simulink model "vv_casper"  (R2013b)
settings: Solver=ode45  StartTime=0.0  StopTime=10.0  RelTol=1e-3
undefined symbols (not defined in the file or in its folder): pfb_coeff_gen_calc
undefined symbols (not defined in the file): xlfda_numerator
libraries: xbsIndex_r4 x17488, casper_library_delays x78, casper_library_misc x51, dspsigops x32, xps_library x3, xbsReplacements_r4 x2
(part 7 of 164)

== system vv_casper/dec_fir ==
  sync_in : Inport
  real1 : Inport  Port=2
  imag1 : Inport  Port=3
  real2 : Inport  Port=4
  imag2 : Inport  Port=5
  real3 : Inport  Port=6
  imag3 : Inport  Port=7
  real4 : Inport  Port=8
  imag4 : Inport  Port=9
  real5 : Inport  Port=10
  imag5 : Inport  Port=11
  real6 : Inport  Port=12
  imag6 : Inport  Port=13
  real7 : Inport  Port=14
  imag7 : Inport  Port=15
  real8 : Inport  Port=16
  imag8 : Inport  Port=17
  real9 : Inport  Port=18
  imag9 : Inport  Port=19
  real10 : Inport  Port=20
  imag10 : Inport  Port=21
  real11 : Inport  Port=22
  imag11 : Inport  Port=23
  real12 : Inport  Port=24
  imag12 : Inport  Port=25
  real13 : Inport  Port=26
  imag13 : Inport  Port=27
  real14 : Inport  Port=28
  imag14 : Inport  Port=29
  real15 : Inport  Port=30
  imag15 : Inport  Port=31
  real16 : Inport  Port=32
  imag16 : Inport  Port=33
  convert1 : xbsIndex_r4/Convert  gui_display_data_type=Fixed-point  arith_type="Signed  (2's comp)"  n_bits=35  bin_pt=34  float_type=Single  exp_bits=8  fraction_bits=24  quantization="Round  (unbiased: +/- Inf)"  overflow=Wrap  en=off  latency=2  dbl_ovrd=off  pipeline=off  block_type=convert
  convert2 : xbsIndex_r4/Convert  gui_display_data_type=Fixed-point  arith_type="Signed  (2's comp)"  n_bits=35  bin_pt=34  float_type=Single  exp_bits=8  fraction_bits=24  quantization="Round  (unbiased: +/- Inf)"  overflow=Wrap  en=off  latency=2  dbl_ovrd=off  pipeline=off  block_type=convert
  delay : xbsIndex_r4/Delay  rst=off  infoeditControl=Selection of Reset will increase slice count due to use of real FFs and instead of SRLs  en=off  latency=9  dbl_ovrd=off  reg_retiming=off  block_type=delay
  fir_dbl_col1 : Subsystem  AncestorBlock=casper_library_downconverter/fir_dbl_col  mask(fir_dbl_col){n_inputs=16, coeff=[-0.00011716 -9.1991e-05 -6.4266e-05  -3.536e-05 -6.6251e-06  2.0662e-05  4.5356e-05  6.6484e-05  8.3286e-05  9.5227e-05  0.00010202  0.00010362   0.0001002   9.217e-05  8.0098e-05  6.4705e-05], add_latency=1, mult_latency=2, coeff_bit_width=25, coeff_bin_pt=24, first_stage_hdl=on, adder_imp=DSP48}
      mask prompts: n_inputs "Inputs"; coeff "Coefficients"; add_latency "Add latency"; mult_latency "Mult Latency"; coeff_bit_width "Coefficient bit width"; coeff_bin_pt "Coefficient binary point"; first_stage_hdl "Implement first stage of adder trees on output as behavioural HDL"; adder_imp "Adder implementation"
      mask init:
      | fir_dbl_col_init(gcb, ...
      |     'n_inputs', n_inputs, ...
      |     'coeff', coeff, ...
      |     'mult_latency', mult_latency, ...
      |     'add_latency', add_latency, ...
      |     'coeff_bit_width', coeff_bit_width, ...
      |     'coeff_bin_pt', coeff_bin_pt,  ...
      |     'first_stage_hdl', first_stage_hdl, ...
      |     'adder_imp', adder_imp);
      mask Help: eval('xlWeb(''http://casper.berkeley.edu/wiki/Fir_dbl_col'')')
      mask TypeOptions adder_imp: Behavioral | Fabric | DSP48
  fir_dbl_col10 : Subsystem  AncestorBlock=casper_library_downconverter/fir_dbl_col  mask(fir_dbl_col){n_inputs=16, coeff=[0.0019945   0.0022285   0.0023628   0.0023951   0.0023272   0.0021652   0.0019186   0.0016003   0.0012258  0.00081224    0.000378 -5.8305e-05 -0.00047857 -0.00086589  -0.0012053  -0.0014841], add_latency=1, mult_latency=2, coeff_bit_width=25, coeff_bin_pt=24, first_stage_hdl=on, adder_imp=DSP48}
      mask prompts: n_inputs "Inputs"; coeff "Coefficients"; add_latency "Add latency"; mult_latency "Mult Latency"; coeff_bit_width "Coefficient bit width"; coeff_bin_pt "Coefficient binary point"; first_stage_hdl "Implement first stage of adder trees on output as behavioural HDL"; adder_imp "Adder implementation"
      mask init: same as vv_casper/dec_fir/fir_dbl_col1
      mask Help: eval('xlWeb(''http://casper.berkeley.edu/wiki/Fir_dbl_col'')')
      mask TypeOptions adder_imp: Behavioral | Fabric | DSP48
  fir_dbl_col11 : Subsystem  AncestorBlock=casper_library_downconverter/fir_dbl_col  mask(fir_dbl_col){n_inputs=16, coeff=[-0.0023054  -0.0026857  -0.0029423  -0.0030687  -0.0030641  -0.0029331  -0.0026851  -0.0023343  -0.0018984  -0.0013982 -0.00085648 -0.00029684  0.00025703  0.00078246   0.0012587   0.0016676], add_latency=1, mult_latency=2, coeff_bit_width=25, coeff_bin_pt=24, first_stage_hdl=on, adder_imp=DSP48}
      mask prompts: n_inputs "Inputs"; coeff "Coefficients"; add_latency "Add latency"; mult_latency "Mult Latency"; coeff_bit_width "Coefficient bit width"; coeff_bin_pt "Coefficient binary point"; first_stage_hdl "Implement first stage of adder trees on output as behavioural HDL"; adder_imp "Adder implementation"
      mask init: same as vv_casper/dec_fir/fir_dbl_col1
      mask Help: eval('xlWeb(''http://casper.berkeley.edu/wiki/Fir_dbl_col'')')
      mask TypeOptions adder_imp: Behavioral | Fabric | DSP48
  fir_dbl_col12 : Subsystem  AncestorBlock=casper_library_downconverter/fir_dbl_col  mask(fir_dbl_col){n_inputs=16, coeff=[0.0026286   0.0032244    0.003665   0.0039383   0.0040391   0.0039697   0.0037391   0.0033626   0.0028607   0.0022586   0.0015845  0.00086849   0.0001415 -0.00056625  -0.0012263  -0.0018133], add_latency=1, mult_latency=2, coeff_bit_width=25, coeff_bin_pt=24, first_stage_hdl=on, adder_imp=DSP48}
      mask prompts: n_inputs "Inputs"; coeff "Coefficients"; add_latency "Add latency"; mult_latency "Mult Latency"; coeff_bit_width "Coefficient bit width"; coeff_bin_pt "Coefficient binary point"; first_stage_hdl "Implement first stage of adder trees on output as behavioural HDL"; adder_imp "Adder implementation"
      mask init: same as vv_casper/dec_fir/fir_dbl_col1
      mask Help: eval('xlWeb(''http://casper.berkeley.edu/wiki/Fir_dbl_col'')')
      mask TypeOptions adder_imp: Behavioral | Fabric | DSP48
  fir_dbl_col13 : Subsystem  AncestorBlock=casper_library_downconverter/fir_dbl_col  mask(fir_dbl_col){n_inputs=16, coeff=[-0.0029853  -0.0039218  -0.0046552  -0.0051649  -0.0054403  -0.0054803  -0.0052935  -0.0048969  -0.0043155  -0.0035804  -0.0027279  -0.0017974 -0.00082976  0.00013403   0.0010549   0.0018968], add_latency=1, mult_latency=2, coeff_bit_width=25, coeff_bin_pt=24, first_stage_hdl=on, adder_imp=DSP48}
      mask prompts: n_inputs "Inputs"; coeff "Coefficients"; add_latency "Add latency"; mult_latency "Mult Latency"; coeff_bit_width "Coefficient bit width"; coeff_bin_pt "Coefficient binary point"; first_stage_hdl "Implement first stage of adder trees on output as behavioural HDL"; adder_imp "Adder implementation"
      mask init: same as vv_casper/dec_fir/fir_dbl_col1
      mask Help: eval('xlWeb(''http://casper.berkeley.edu/wiki/Fir_dbl_col'')')
      mask TypeOptions adder_imp: Behavioral | Fabric | DSP48
  fir_dbl_col14 : Subsystem  AncestorBlock=casper_library_downconverter/fir_dbl_col  mask(fir_dbl_col){n_inputs=16, coeff=[0.0034602   0.0050242   0.0062876   0.0072191    0.007802   0.0080335   0.0079243   0.0074975   0.0067875   0.0058373   0.0046975   0.0034231   0.0020719  0.00070185 -0.00063127  -0.0018756], add_latency=1, mult_latency=2, coeff_bit_width=25, coeff_bin_pt=24, first_stage_hdl=on, adder_imp=DSP48}
      mask prompts: n_inputs "Inputs"; coeff "Coefficients"; add_latency "Add latency"; mult_latency "Mult Latency"; coeff_bit_width "Coefficient bit width"; coeff_bin_pt "Coefficient binary point"; first_stage_hdl "Implement first stage of adder trees on output as behavioural HDL"; adder_imp "Adder implementation"
      mask init: same as vv_casper/dec_fir/fir_dbl_col1
      mask Help: eval('xlWeb(''http://casper.berkeley.edu/wiki/Fir_dbl_col'')')
      mask TypeOptions adder_imp: Behavioral | Fabric | DSP48
  fir_dbl_col15 : Subsystem  AncestorBlock=casper_library_downconverter/fir_dbl_col  mask(fir_dbl_col){n_inputs=16, coeff=[-0.004503  -0.0077173   -0.010272   -0.012152    -0.01336   -0.013919    -0.01387   -0.013269   -0.012184   -0.010697  -0.0088951  -0.0068697  -0.0047146  -0.0025212 -0.00037637   0.0016407], add_latency=1, mult_latency=2, coeff_bit_width=25, coeff_bin_pt=24, first_stage_hdl=on, adder_imp=DSP48}
      mask prompts: n_inputs "Inputs"; coeff "Coefficients"; add_latency "Add latency"; mult_latency "Mult Latency"; coeff_bit_width "Coefficient bit width"; coeff_bin_pt "Coefficient binary point"; first_stage_hdl "Implement first stage of adder trees on output as behavioural HDL"; adder_imp "Adder implementation"
      mask init: same as vv_casper/dec_fir/fir_dbl_col1
      mask Help: eval('xlWeb(''http://casper.berkeley.edu/wiki/Fir_dbl_col'')')
      mask TypeOptions adder_imp: Behavioral | Fabric | DSP48
  fir_dbl_col16 : Subsystem  AncestorBlock=casper_library_downconverter/fir_dbl_col  mask(fir_dbl_col){n_inputs=16, coeff=[0.065072    0.064162    0.062365    0.059726    0.056312    0.052207    0.047514    0.042348    0.036834    0.031102    0.025287    0.019521     0.01393    0.008634    0.003738 -0.00066588], add_latency=1, mult_latency=2, coeff_bit_width=25, coeff_bin_pt=24, first_stage_hdl=on, adder_imp=DSP48}
      mask prompts: n_inputs "Inputs"; coeff "Coefficients"; add_latency "Add latency"; mult_latency "Mult Latency"; coeff_bit_width "Coefficient bit width"; coeff_bin_pt "Coefficient binary point"; first_stage_hdl "Implement first stage of adder trees on output as behavioural HDL"; adder_imp "Adder implementation"
      mask init: same as vv_casper/dec_fir/fir_dbl_col1
      mask Help: eval('xlWeb(''http://casper.berkeley.edu/wiki/Fir_dbl_col'')')
      mask TypeOptions adder_imp: Behavioral | Fabric | DSP48
  fir_dbl_col2 : Subsystem  AncestorBlock=casper_library_downconverter/fir_dbl_col  mask(fir_dbl_col){n_inputs=16, coeff=[0.00020848  0.00017636  0.00013837  9.6442e-05  5.2572e-05  8.7473e-06 -3.3147e-05   -7.14e-05 -0.00010455 -0.00013141 -0.00015117 -0.00016332 -0.00016775 -0.00016468 -0.00015464 -0.00013845], add_latency=1, mult_latency=2, coeff_bit_width=25, coeff_bin_pt=24, first_stage_hdl=on, adder_imp=DSP48}
      mask prompts: n_inputs "Inputs"; coeff "Coefficients"; add_latency "Add latency"; mult_latency "Mult Latency"; coeff_bit_width "Coefficient bit width"; coeff_bin_pt "Coefficient binary point"; first_stage_hdl "Implement first stage of adder trees on output as behavioural HDL"; adder_imp "Adder implementation"
      mask init: same as vv_casper/dec_fir/fir_dbl_col1
      mask Help: eval('xlWeb(''http://casper.berkeley.edu/wiki/Fir_dbl_col'')')
      mask TypeOptions adder_imp: Behavioral | Fabric | DSP48
  fir_dbl_col3 : Subsystem  AncestorBlock=casper_library_downconverter/fir_dbl_col  mask(fir_dbl_col){n_inputs=16, coeff=[-0.00032924 -0.00029221 -0.00024455 -0.00018874 -0.00012752 -6.3715e-05  -1.479e-07  6.0493e-05  0.00011577  0.00016357  0.00020222  0.00023048  0.00024766  0.00025353   0.0002484  0.00023299], add_latency=1, mult_latency=2, coeff_bit_width=25, coeff_bin_pt=24, first_stage_hdl=on, adder_imp=DSP48}
      mask prompts: n_inputs "Inputs"; coeff "Coefficients"; add_latency "Add latency"; mult_latency "Mult Latency"; coeff_bit_width "Coefficient bit width"; coeff_bin_pt "Coefficient binary point"; first_stage_hdl "Implement first stage of adder trees on output as behavioural HDL"; adder_imp "Adder implementation"
      mask init: same as vv_casper/dec_fir/fir_dbl_col1
      mask Help: eval('xlWeb(''http://casper.berkeley.edu/wiki/Fir_dbl_col'')')
      mask TypeOptions adder_imp: Behavioral | Fabric | DSP48
  fir_dbl_col4 : Subsystem  AncestorBlock=casper_library_downconverter/fir_dbl_col  mask(fir_dbl_col){n_inputs=16, coeff=[0.00048235  0.00044471  0.00038999  0.00032117   0.0002417  0.00015536  6.6049e-05 -2.2349e-05 -0.00010615 -0.00018201 -0.00024707 -0.00029904 -0.00033626 -0.00035779  -0.0003634 -0.00035352], add_latency=1, mult_latency=2, coeff_bit_width=25, coeff_bin_pt=24, first_stage_hdl=on, adder_imp=DSP48}
      mask prompts: n_inputs "Inputs"; coeff "Coefficients"; add_latency "Add latency"; mult_latency "Mult Latency"; coeff_bit_width "Coefficient bit width"; coeff_bin_pt "Coefficient binary point"; first_stage_hdl "Implement first stage of adder trees on output as behavioural HDL"; adder_imp "Adder implementation"
      mask init: same as vv_casper/dec_fir/fir_dbl_col1
      mask Help: eval('xlWeb(''http://casper.berkeley.edu/wiki/Fir_dbl_col'')')
      mask TypeOptions adder_imp: Behavioral | Fabric | DSP48
  fir_dbl_col5 : Subsystem  AncestorBlock=casper_library_downconverter/fir_dbl_col  mask(fir_dbl_col){n_inputs=16, coeff=[-0.00066852 -0.00063712 -0.00058034 -0.00050146  -0.0004046 -0.00029448 -0.00017619 -5.4992e-05  6.3927e-05  0.00017567  0.00027583  0.00036064  0.00042714  0.00047323  0.00049777  0.00050057], add_latency=1, mult_latency=2, coeff_bit_width=25, coeff_bin_pt=24, first_stage_hdl=on, adder_imp=DSP48}
      mask prompts: n_inputs "Inputs"; coeff "Coefficients"; add_latency "Add latency"; mult_latency "Mult Latency"; coeff_bit_width "Coefficient bit width"; coeff_bin_pt "Coefficient binary point"; first_stage_hdl "Implement first stage of adder trees on output as behavioural HDL"; adder_imp "Adder implementation"
      mask init: same as vv_casper/dec_fir/fir_dbl_col1
      mask Help: eval('xlWeb(''http://casper.berkeley.edu/wiki/Fir_dbl_col'')')
      mask TypeOptions adder_imp: Behavioral | Fabric | DSP48
  fir_dbl_col6 : Subsystem  AncestorBlock=casper_library_downconverter/fir_dbl_col  mask(fir_dbl_col){n_inputs=16, coeff=[0.00088649   0.0008712  0.00082022  0.00073687  0.00062575  0.00049244  0.00034327  0.00018502  2.4603e-05  -0.0001312 -0.00027605 -0.00040428 -0.00051111 -0.00059285 -0.00064697  -0.0006722], add_latency=1, mult_latency=2, coeff_bit_width=25, coeff_bin_pt=24, first_stage_hdl=on, adder_imp=DSP48}
      mask prompts: n_inputs "Inputs"; coeff "Coefficients"; add_latency "Add latency"; mult_latency "Mult Latency"; coeff_bit_width "Coefficient bit width"; coeff_bin_pt "Coefficient binary point"; first_stage_hdl "Implement first stage of adder trees on output as behavioural HDL"; adder_imp "Adder implementation"
      mask init: same as vv_casper/dec_fir/fir_dbl_col1
      mask Help: eval('xlWeb(''http://casper.berkeley.edu/wiki/Fir_dbl_col'')')
      mask TypeOptions adder_imp: Behavioral | Fabric | DSP48
  fir_dbl_col7 : Subsystem  AncestorBlock=casper_library_downconverter/fir_dbl_col  mask(fir_dbl_col){n_inputs=16, coeff=[-0.0011332  -0.0011474  -0.0011135  -0.0010345 -0.00091512 -0.00076162 -0.00058152  -0.0003832  -0.0001755  3.2606e-05  0.00023245  0.00041597  0.00057606  0.00070685  0.00080384  0.00086415], add_latency=1, mult_latency=2, coeff_bit_width=25, coeff_bin_pt=24, first_stage_hdl=on, adder_imp=DSP48}
      mask prompts: n_inputs "Inputs"; coeff "Coefficients"; add_latency "Add latency"; mult_latency "Mult Latency"; coeff_bit_width "Coefficient bit width"; coeff_bin_pt "Coefficient binary point"; first_stage_hdl "Implement first stage of adder trees on output as behavioural HDL"; adder_imp "Adder implementation"
      mask init: same as vv_casper/dec_fir/fir_dbl_col1
      mask Help: eval('xlWeb(''http://casper.berkeley.edu/wiki/Fir_dbl_col'')')
      mask TypeOptions adder_imp: Behavioral | Fabric | DSP48
  fir_dbl_col8 : Subsystem  AncestorBlock=casper_library_downconverter/fir_dbl_col  mask(fir_dbl_col){n_inputs=16, coeff=[0.0014038   0.0014653   0.0014641   0.0014022    0.001284   0.0011164  0.00090766  0.00066792  0.00040807  0.00013955 -0.00012621 -0.00037824 -0.00060651 -0.00080228 -0.00095846  -0.0010698], add_latency=1, mult_latency=2, coeff_bit_width=25, coeff_bin_pt=24, first_stage_hdl=on, adder_imp=DSP48}
      mask prompts: n_inputs "Inputs"; coeff "Coefficients"; add_latency "Add latency"; mult_latency "Mult Latency"; coeff_bit_width "Coefficient bit width"; coeff_bin_pt "Coefficient binary point"; first_stage_hdl "Implement first stage of adder trees on output as behavioural HDL"; adder_imp "Adder implementation"
      mask init: same as vv_casper/dec_fir/fir_dbl_col1
      mask Help: eval('xlWeb(''http://casper.berkeley.edu/wiki/Fir_dbl_col'')')
      mask TypeOptions adder_imp: Behavioral | Fabric | DSP48
  fir_dbl_col9 : Subsystem  AncestorBlock=casper_library_downconverter/fir_dbl_col  mask(fir_dbl_col){n_inputs=16, coeff=[-0.0016928  -0.0018249  -0.0018772  -0.0018501  -0.0017472  -0.0015751  -0.0013431  -0.0010626 -0.00074681 -0.00040991 -6.6527e-05   0.0002689   0.0005827  0.00086252   0.0010978   0.0012802], add_latency=1, mult_latency=2, coeff_bit_width=25, coeff_bin_pt=24, first_stage_hdl=on, adder_imp=DSP48}
      mask prompts: n_inputs "Inputs"; coeff "Coefficients"; add_latency "Add latency"; mult_latency "Mult Latency"; coeff_bit_width "Coefficient bit width"; coeff_bin_pt "Coefficient binary point"; first_stage_hdl "Implement first stage of adder trees on output as behavioural HDL"; adder_imp "Adder implementation"
      mask init: same as vv_casper/dec_fir/fir_dbl_col1
      mask Help: eval('xlWeb(''http://casper.berkeley.edu/wiki/Fir_dbl_col'')')
      mask TypeOptions adder_imp: Behavioral | Fabric | DSP48
  imag_sum : Subsystem  AncestorBlock=casper_library_misc/adder_tree  mask(adder_tree){n_inputs=16, latency=1, adder_imp=DSP48, first_stage_hdl=off}
      mask prompts: n_inputs "Number of Inputs"; latency "Add Latency"; adder_imp "Adder implementation"; first_stage_hdl "Use behavioural HDL for first stage of adders"
      mask help:
      | Sums all inputs using a tree of adds and delays.
      |
      | Number of inputs: The number of inputs to the block to be summed
      | Add latency: The number of clock cycles to perform one addition (affects timing)..
      | Adder implementation: choice of fabric or DSP48E core, or behavioral HDL
      | Use behavioural HDL for first stage of adders: Causes the first stage of adders to be absorbed into DSP blocks if multipliers precede them (Virtex 5). Overrides Adder implementation
      mask init:
      | adder_tree_init(gcb, ...
      |     'n_inputs', n_inputs, ...
      |     'latency', latency, ...
      |     'adder_imp', adder_imp, ...
      |     'first_stage_hdl', first_stage_hdl);
      settings: AttributesFormatString=latency 4
      mask Help: eval('xlWeb(''http://casper.berkeley.edu/wiki/Adder_tree'')')
      mask TypeOptions adder_imp: Behavioral | Fabric | DSP48
  real_sum : Subsystem  AncestorBlock=casper_library_misc/adder_tree  mask(adder_tree){n_inputs=16, latency=1, adder_imp=DSP48, first_stage_hdl=off}
      mask prompts: n_inputs "Number of Inputs"; latency "Add Latency"; adder_imp "Adder implementation"; first_stage_hdl "Use behavioural HDL for first stage of adders"
      mask help:
      | Sums all inputs using a tree of adds and delays.
      |
      | Number of inputs: The number of inputs to the block to be summed
      | Add latency: The number of clock cycles to perform one addition (affects timing)..
      | Adder implementation: choice of fabric or DSP48E core, or behavioral HDL
      | Use behavioural HDL for first stage of adders: Causes the first stage of adders to be absorbed into DSP blocks if multipliers precede them (Virtex 5). Overrides Adder implementation
      mask init:
      | adder_tree_init(gcb, ...
      |     'n_inputs', n_inputs, ...
      |     'latency', latency, ...
      |     'adder_imp', adder_imp, ...
      |     'first_stage_hdl', first_stage_hdl);
      settings: AttributesFormatString=latency 4
      mask Help: eval('xlWeb(''http://casper.berkeley.edu/wiki/Adder_tree'')')
      mask TypeOptions adder_imp: Behavioral | Fabric | DSP48
  ri_to_c : casper_library_misc/ri_to_c
  shift1 : xbsIndex_r4/Shift  shift_dir=Left  shift_bits=0  en=off  latency=0  precision=Full  arith_type="Signed  (2's comp)"  n_bits=16  bin_pt=14  quantization=Truncate  overflow=Wrap  dbl_ovrd=off  block_type=shift
  shift2 : xbsIndex_r4/Shift  shift_dir=Left  shift_bits=0  en=off  latency=0  precision=Full  arith_type="Signed  (2's comp)"  n_bits=16  bin_pt=14  quantization=Truncate  overflow=Wrap  dbl_ovrd=off  block_type=shift
  sync_out : Outport
  dout : Outport  Port=2
  wires:
  real1/1 -> fir_dbl_col1/1(real1)
  imag1/1 -> fir_dbl_col1/2(imag1)
  real2/1 -> fir_dbl_col1/3(real2)
  imag2/1 -> fir_dbl_col1/4(imag2)
  real3/1 -> fir_dbl_col1/5(real3)
  imag3/1 -> fir_dbl_col1/6(imag3)
  real4/1 -> fir_dbl_col1/7(real4)
  imag4/1 -> fir_dbl_col1/8(imag4)
  real5/1 -> fir_dbl_col1/9(real5)
  imag5/1 -> fir_dbl_col1/10(imag5)
  real6/1 -> fir_dbl_col1/11(real6)
  imag6/1 -> fir_dbl_col1/12(imag6)
  real7/1 -> fir_dbl_col1/13(real7)
  imag7/1 -> fir_dbl_col1/14(imag7)
  real8/1 -> fir_dbl_col1/15(real8)
  imag8/1 -> fir_dbl_col1/16(imag8)
  real9/1 -> fir_dbl_col1/17(real9)
  imag9/1 -> fir_dbl_col1/18(imag9)
  real10/1 -> fir_dbl_col1/19(real10)
  imag10/1 -> fir_dbl_col1/20(imag10)
  real11/1 -> fir_dbl_col1/21(real11)
  imag11/1 -> fir_dbl_col1/22(imag11)
  real12/1 -> fir_dbl_col1/23(real12)
  imag12/1 -> fir_dbl_col1/24(imag12)
  real13/1 -> fir_dbl_col1/25(real13)
  imag13/1 -> fir_dbl_col1/26(imag13)
  real14/1 -> fir_dbl_col1/27(real14)
  imag14/1 -> fir_dbl_col1/28(imag14)
  real15/1 -> fir_dbl_col1/29(real15)
  imag15/1 -> fir_dbl_col1/30(imag15)
  real16/1 -> fir_dbl_col1/31(real16)
  imag16/1 -> fir_dbl_col1/32(imag16)
  fir_dbl_col1/65(real_sum) -> real_sum/2(din1)
  fir_dbl_col1/66(imag_sum) -> imag_sum/2(din1)
  fir_dbl_col1/1(real_out1) -> fir_dbl_col2/1(real1)
  fir_dbl_col1/2(imag_out1) -> fir_dbl_col2/2(imag1)
  fir_dbl_col1/3(real_out2) -> fir_dbl_col2/3(real2)
  fir_dbl_col1/4(imag_out2) -> fir_dbl_col2/4(imag2)
  fir_dbl_col1/5(real_out3) -> fir_dbl_col2/5(real3)
  fir_dbl_col1/6(imag_out3) -> fir_dbl_col2/6(imag3)
  fir_dbl_col1/7(real_out4) -> fir_dbl_col2/7(real4)
  fir_dbl_col1/8(imag_out4) -> fir_dbl_col2/8(imag4)
  fir_dbl_col1/9(real_out5) -> fir_dbl_col2/9(real5)
  fir_dbl_col1/10(imag_out5) -> fir_dbl_col2/10(imag5)
  fir_dbl_col1/11(real_out6) -> fir_dbl_col2/11(real6)
  fir_dbl_col1/12(imag_out6) -> fir_dbl_col2/12(imag6)
  fir_dbl_col1/13(real_out7) -> fir_dbl_col2/13(real7)
  fir_dbl_col1/14(imag_out7) -> fir_dbl_col2/14(imag7)
  fir_dbl_col1/15(real_out8) -> fir_dbl_col2/15(real8)
  fir_dbl_col1/16(imag_out8) -> fir_dbl_col2/16(imag8)
  fir_dbl_col1/17(real_out9) -> fir_dbl_col2/17(real9)
  fir_dbl_col1/18(imag_out9) -> fir_dbl_col2/18(imag9)
  fir_dbl_col1/19(real_out10) -> fir_dbl_col2/19(real10)
  fir_dbl_col1/20(imag_out10) -> fir_dbl_col2/20(imag10)
  fir_dbl_col1/21(real_out11) -> fir_dbl_col2/21(real11)
  fir_dbl_col1/22(imag_out11) -> fir_dbl_col2/22(imag11)
  fir_dbl_col1/23(real_out12) -> fir_dbl_col2/23(real12)
  fir_dbl_col1/24(imag_out12) -> fir_dbl_col2/24(imag12)
  fir_dbl_col1/25(real_out13) -> fir_dbl_col2/25(real13)
  fir_dbl_col1/26(imag_out13) -> fir_dbl_col2/26(imag13)
  fir_dbl_col1/27(real_out14) -> fir_dbl_col2/27(real14)
  fir_dbl_col1/28(imag_out14) -> fir_dbl_col2/28(imag14)
  fir_dbl_col1/29(real_out15) -> fir_dbl_col2/29(real15)
  fir_dbl_col1/30(imag_out15) -> fir_dbl_col2/30(imag15)
  fir_dbl_col1/31(real_out16) -> fir_dbl_col2/31(real16)
  fir_dbl_col1/32(imag_out16) -> fir_dbl_col2/32(imag16)
  fir_dbl_col2/65(real_sum) -> real_sum/3(din2)
  fir_dbl_col2/66(imag_sum) -> imag_sum/3(din2)
  fir_dbl_col2/1(real_out1) -> fir_dbl_col3/1(real1)
  fir_dbl_col2/2(imag_out1) -> fir_dbl_col3/2(imag1)
  fir_dbl_col2/3(real_out2) -> fir_dbl_col3/3(real2)
  fir_dbl_col2/4(imag_out2) -> fir_dbl_col3/4(imag2)
  fir_dbl_col2/5(real_out3) -> fir_dbl_col3/5(real3)
  fir_dbl_col2/6(imag_out3) -> fir_dbl_col3/6(imag3)
  fir_dbl_col2/7(real_out4) -> fir_dbl_col3/7(real4)
  fir_dbl_col2/8(imag_out4) -> fir_dbl_col3/8(imag4)
  fir_dbl_col2/9(real_out5) -> fir_dbl_col3/9(real5)
  fir_dbl_col2/10(imag_out5) -> fir_dbl_col3/10(imag5)
  fir_dbl_col2/11(real_out6) -> fir_dbl_col3/11(real6)
  fir_dbl_col2/12(imag_out6) -> fir_dbl_col3/12(imag6)
  fir_dbl_col2/13(real_out7) -> fir_dbl_col3/13(real7)
  fir_dbl_col2/14(imag_out7) -> fir_dbl_col3/14(imag7)
  fir_dbl_col2/15(real_out8) -> fir_dbl_col3/15(real8)
  fir_dbl_col2/16(imag_out8) -> fir_dbl_col3/16(imag8)
  fir_dbl_col2/17(real_out9) -> fir_dbl_col3/17(real9)
  fir_dbl_col2/18(imag_out9) -> fir_dbl_col3/18(imag9)
  fir_dbl_col2/19(real_out10) -> fir_dbl_col3/19(real10)
  fir_dbl_col2/20(imag_out10) -> fir_dbl_col3/20(imag10)
  fir_dbl_col2/21(real_out11) -> fir_dbl_col3/21(real11)
  fir_dbl_col2/22(imag_out11) -> fir_dbl_col3/22(imag11)
  fir_dbl_col2/23(real_out12) -> fir_dbl_col3/23(real12)
  fir_dbl_col2/24(imag_out12) -> fir_dbl_col3/24(imag12)
  fir_dbl_col2/25(real_out13) -> fir_dbl_col3/25(real13)
  fir_dbl_col2/26(imag_out13) -> fir_dbl_col3/26(imag13)
  fir_dbl_col2/27(real_out14) -> fir_dbl_col3/27(real14)
  fir_dbl_col2/28(imag_out14) -> fir_dbl_col3/28(imag14)
  fir_dbl_col2/29(real_out15) -> fir_dbl_col3/29(real15)
  fir_dbl_col2/30(imag_out15) -> fir_dbl_col3/30(imag15)
  fir_dbl_col2/31(real_out16) -> fir_dbl_col3/31(real16)
  fir_dbl_col2/32(imag_out16) -> fir_dbl_col3/32(imag16)
  fir_dbl_col3/65(real_sum) -> real_sum/4(din3)
  fir_dbl_col3/66(imag_sum) -> imag_sum/4(din3)
  fir_dbl_col3/1(real_out1) -> fir_dbl_col4/1(real1)
  fir_dbl_col3/2(imag_out1) -> fir_dbl_col4/2(imag1)
  fir_dbl_col3/3(real_out2) -> fir_dbl_col4/3(real2)
  fir_dbl_col3/4(imag_out2) -> fir_dbl_col4/4(imag2)
  fir_dbl_col3/5(real_out3) -> fir_dbl_col4/5(real3)
  fir_dbl_col3/6(imag_out3) -> fir_dbl_col4/6(imag3)
  fir_dbl_col3/7(real_out4) -> fir_dbl_col4/7(real4)
  fir_dbl_col3/8(imag_out4) -> fir_dbl_col4/8(imag4)
  fir_dbl_col3/9(real_out5) -> fir_dbl_col4/9(real5)
  fir_dbl_col3/10(imag_out5) -> fir_dbl_col4/10(imag5)
  fir_dbl_col3/11(real_out6) -> fir_dbl_col4/11(real6)
  fir_dbl_col3/12(imag_out6) -> fir_dbl_col4/12(imag6)
  fir_dbl_col3/13(real_out7) -> fir_dbl_col4/13(real7)
  fir_dbl_col3/14(imag_out7) -> fir_dbl_col4/14(imag7)
  fir_dbl_col3/15(real_out8) -> fir_dbl_col4/15(real8)
  fir_dbl_col3/16(imag_out8) -> fir_dbl_col4/16(imag8)
  fir_dbl_col3/17(real_out9) -> fir_dbl_col4/17(real9)
  fir_dbl_col3/18(imag_out9) -> fir_dbl_col4/18(imag9)
  fir_dbl_col3/19(real_out10) -> fir_dbl_col4/19(real10)
  fir_dbl_col3/20(imag_out10) -> fir_dbl_col4/20(imag10)
  fir_dbl_col3/21(real_out11) -> fir_dbl_col4/21(real11)
  fir_dbl_col3/22(imag_out11) -> fir_dbl_col4/22(imag11)
  fir_dbl_col3/23(real_out12) -> fir_dbl_col4/23(real12)
  fir_dbl_col3/24(imag_out12) -> fir_dbl_col4/24(imag12)
  fir_dbl_col3/25(real_out13) -> fir_dbl_col4/25(real13)
  fir_dbl_col3/26(imag_out13) -> fir_dbl_col4/26(imag13)
  fir_dbl_col3/27(real_out14) -> fir_dbl_col4/27(real14)
  fir_dbl_col3/28(imag_out14) -> fir_dbl_col4/28(imag14)
  fir_dbl_col3/29(real_out15) -> fir_dbl_col4/29(real15)
  fir_dbl_col3/30(imag_out15) -> fir_dbl_col4/30(imag15)
  fir_dbl_col3/31(real_out16) -> fir_dbl_col4/31(real16)
  fir_dbl_col3/32(imag_out16) -> fir_dbl_col4/32(imag16)
  fir_dbl_col4/65(real_sum) -> real_sum/5(din4)
  fir_dbl_col4/66(imag_sum) -> imag_sum/5(din4)
  fir_dbl_col4/1(real_out1) -> fir_dbl_col5/1(real1)
  fir_dbl_col4/2(imag_out1) -> fir_dbl_col5/2(imag1)
  fir_dbl_col4/3(real_out2) -> fir_dbl_col5/3(real2)
  fir_dbl_col4/4(imag_out2) -> fir_dbl_col5/4(imag2)
  fir_dbl_col4/5(real_out3) -> fir_dbl_col5/5(real3)
  fir_dbl_col4/6(imag_out3) -> fir_dbl_col5/6(imag3)
  fir_dbl_col4/7(real_out4) -> fir_dbl_col5/7(real4)
  fir_dbl_col4/8(imag_out4) -> fir_dbl_col5/8(imag4)
  fir_dbl_col4/9(real_out5) -> fir_dbl_col5/9(real5)
  fir_dbl_col4/10(imag_out5) -> fir_dbl_col5/10(imag5)
  fir_dbl_col4/11(real_out6) -> fir_dbl_col5/11(real6)
  fir_dbl_col4/12(imag_out6) -> fir_dbl_col5/12(imag6)
  fir_dbl_col4/13(real_out7) -> fir_dbl_col5/13(real7)
  fir_dbl_col4/14(imag_out7) -> fir_dbl_col5/14(imag7)
  fir_dbl_col4/15(real_out8) -> fir_dbl_col5/15(real8)
  fir_dbl_col4/16(imag_out8) -> fir_dbl_col5/16(imag8)
  fir_dbl_col4/17(real_out9) -> fir_dbl_col5/17(real9)
  fir_dbl_col4/18(imag_out9) -> fir_dbl_col5/18(imag9)
  fir_dbl_col4/19(real_out10) -> fir_dbl_col5/19(real10)
  fir_dbl_col4/20(imag_out10) -> fir_dbl_col5/20(imag10)
  fir_dbl_col4/21(real_out11) -> fir_dbl_col5/21(real11)
  fir_dbl_col4/22(imag_out11) -> fir_dbl_col5/22(imag11)
  fir_dbl_col4/23(real_out12) -> fir_dbl_col5/23(real12)
  fir_dbl_col4/24(imag_out12) -> fir_dbl_col5/24(imag12)
  fir_dbl_col4/25(real_out13) -> fir_dbl_col5/25(real13)
  fir_dbl_col4/26(imag_out13) -> fir_dbl_col5/26(imag13)
  fir_dbl_col4/27(real_out14) -> fir_dbl_col5/27(real14)
  fir_dbl_col4/28(imag_out14) -> fir_dbl_col5/28(imag14)
  fir_dbl_col4/29(real_out15) -> fir_dbl_col5/29(real15)
  fir_dbl_col4/30(imag_out15) -> fir_dbl_col5/30(imag15)
  fir_dbl_col4/31(real_out16) -> fir_dbl_col5/31(real16)
  fir_dbl_col4/32(imag_out16) -> fir_dbl_col5/32(imag16)
  fir_dbl_col5/65(real_sum) -> real_sum/6(din5)
  fir_dbl_col5/66(imag_sum) -> imag_sum/6(din5)
  fir_dbl_col5/1(real_out1) -> fir_dbl_col6/1(real1)
  fir_dbl_col5/2(imag_out1) -> fir_dbl_col6/2(imag1)
  fir_dbl_col5/3(real_out2) -> fir_dbl_col6/3(real2)
  fir_dbl_col5/4(imag_out2) -> fir_dbl_col6/4(imag2)
  fir_dbl_col5/5(real_out3) -> fir_dbl_col6/5(real3)
  fir_dbl_col5/6(imag_out3) -> fir_dbl_col6/6(imag3)
  fir_dbl_col5/7(real_out4) -> fir_dbl_col6/7(real4)
  fir_dbl_col5/8(imag_out4) -> fir_dbl_col6/8(imag4)
  fir_dbl_col5/9(real_out5) -> fir_dbl_col6/9(real5)
  fir_dbl_col5/10(imag_out5) -> fir_dbl_col6/10(imag5)
  fir_dbl_col5/11(real_out6) -> fir_dbl_col6/11(real6)
  fir_dbl_col5/12(imag_out6) -> fir_dbl_col6/12(imag6)
  fir_dbl_col5/13(real_out7) -> fir_dbl_col6/13(real7)
  fir_dbl_col5/14(imag_out7) -> fir_dbl_col6/14(imag7)
  fir_dbl_col5/15(real_out8) -> fir_dbl_col6/15(real8)
  fir_dbl_col5/16(imag_out8) -> fir_dbl_col6/16(imag8)
  fir_dbl_col5/17(real_out9) -> fir_dbl_col6/17(real9)
  fir_dbl_col5/18(imag_out9) -> fir_dbl_col6/18(imag9)
  fir_dbl_col5/19(real_out10) -> fir_dbl_col6/19(real10)
  fir_dbl_col5/20(imag_out10) -> fir_dbl_col6/20(imag10)
  fir_dbl_col5/21(real_out11) -> fir_dbl_col6/21(real11)
  fir_dbl_col5/22(imag_out11) -> fir_dbl_col6/22(imag11)
  fir_dbl_col5/23(real_out12) -> fir_dbl_col6/23(real12)
  fir_dbl_col5/24(imag_out12) -> fir_dbl_col6/24(imag12)
  fir_dbl_col5/25(real_out13) -> fir_dbl_col6/25(real13)
  fir_dbl_col5/26(imag_out13) -> fir_dbl_col6/26(imag13)
  fir_dbl_col5/27(real_out14) -> fir_dbl_col6/27(real14)
  fir_dbl_col5/28(imag_out14) -> fir_dbl_col6/28(imag14)
  fir_dbl_col5/29(real_out15) -> fir_dbl_col6/29(real15)
  fir_dbl_col5/30(imag_out15) -> fir_dbl_col6/30(imag15)
  fir_dbl_col5/31(real_out16) -> fir_dbl_col6/31(real16)
  fir_dbl_col5/32(imag_out16) -> fir_dbl_col6/32(imag16)
  fir_dbl_col6/65(real_sum) -> real_sum/7(din6)
  fir_dbl_col6/66(imag_sum) -> imag_sum/7(din6)
  fir_dbl_col6/1(real_out1) -> fir_dbl_col7/1(real1)
  fir_dbl_col6/2(imag_out1) -> fir_dbl_col7/2(imag1)
  fir_dbl_col6/3(real_out2) -> fir_dbl_col7/3(real2)
  fir_dbl_col6/4(imag_out2) -> fir_dbl_col7/4(imag2)
  fir_dbl_col6/5(real_out3) -> fir_dbl_col7/5(real3)
  fir_dbl_col6/6(imag_out3) -> fir_dbl_col7/6(imag3)
  fir_dbl_col6/7(real_out4) -> fir_dbl_col7/7(real4)
  fir_dbl_col6/8(imag_out4) -> fir_dbl_col7/8(imag4)
  fir_dbl_col6/9(real_out5) -> fir_dbl_col7/9(real5)
  fir_dbl_col6/10(imag_out5) -> fir_dbl_col7/10(imag5)
  fir_dbl_col6/11(real_out6) -> fir_dbl_col7/11(real6)
  fir_dbl_col6/12(imag_out6) -> fir_dbl_col7/12(imag6)
  fir_dbl_col6/13(real_out7) -> fir_dbl_col7/13(real7)
  fir_dbl_col6/14(imag_out7) -> fir_dbl_col7/14(imag7)
  fir_dbl_col6/15(real_out8) -> fir_dbl_col7/15(real8)
  fir_dbl_col6/16(imag_out8) -> fir_dbl_col7/16(imag8)
  fir_dbl_col6/17(real_out9) -> fir_dbl_col7/17(real9)
  fir_dbl_col6/18(imag_out9) -> fir_dbl_col7/18(imag9)
  fir_dbl_col6/19(real_out10) -> fir_dbl_col7/19(real10)
  fir_dbl_col6/20(imag_out10) -> fir_dbl_col7/20(imag10)
  fir_dbl_col6/21(real_out11) -> fir_dbl_col7/21(real11)
  fir_dbl_col6/22(imag_out11) -> fir_dbl_col7/22(imag11)
  fir_dbl_col6/23(real_out12) -> fir_dbl_col7/23(real12)
  fir_dbl_col6/24(imag_out12) -> fir_dbl_col7/24(imag12)
  fir_dbl_col6/25(real_out13) -> fir_dbl_col7/25(real13)
  fir_dbl_col6/26(imag_out13) -> fir_dbl_col7/26(imag13)
  fir_dbl_col6/27(real_out14) -> fir_dbl_col7/27(real14)
  fir_dbl_col6/28(imag_out14) -> fir_dbl_col7/28(imag14)
  fir_dbl_col6/29(real_out15) -> fir_dbl_col7/29(real15)
  fir_dbl_col6/30(imag_out15) -> fir_dbl_col7/30(imag15)
  fir_dbl_col6/31(real_out16) -> fir_dbl_col7/31(real16)
  fir_dbl_col6/32(imag_out16) -> fir_dbl_col7/32(imag16)
  fir_dbl_col7/65(real_sum) -> real_sum/8(din7)
  fir_dbl_col7/66(imag_sum) -> imag_sum/8(din7)
  fir_dbl_col7/1(real_out1) -> fir_dbl_col8/1(real1)
  fir_dbl_col7/2(imag_out1) -> fir_dbl_col8/2(imag1)
  fir_dbl_col7/3(real_out2) -> fir_dbl_col8/3(real2)
  fir_dbl_col7/4(imag_out2) -> fir_dbl_col8/4(imag2)
  fir_dbl_col7/5(real_out3) -> fir_dbl_col8/5(real3)
  fir_dbl_col7/6(imag_out3) -> fir_dbl_col8/6(imag3)
  fir_dbl_col7/7(real_out4) -> fir_dbl_col8/7(real4)
  fir_dbl_col7/8(imag_out4) -> fir_dbl_col8/8(imag4)
  fir_dbl_col7/9(real_out5) -> fir_dbl_col8/9(real5)
  fir_dbl_col7/10(imag_out5) -> fir_dbl_col8/10(imag5)
  fir_dbl_col7/11(real_out6) -> fir_dbl_col8/11(real6)
  fir_dbl_col7/12(imag_out6) -> fir_dbl_col8/12(imag6)
  fir_dbl_col7/13(real_out7) -> fir_dbl_col8/13(real7)
  fir_dbl_col7/14(imag_out7) -> fir_dbl_col8/14(imag7)
  fir_dbl_col7/15(real_out8) -> fir_dbl_col8/15(real8)
  fir_dbl_col7/16(imag_out8) -> fir_dbl_col8/16(imag8)
  fir_dbl_col7/17(real_out9) -> fir_dbl_col8/17(real9)
  fir_dbl_col7/18(imag_out9) -> fir_dbl_col8/18(imag9)
  fir_dbl_col7/19(real_out10) -> fir_dbl_col8/19(real10)
  fir_dbl_col7/20(imag_out10) -> fir_dbl_col8/20(imag10)
  fir_dbl_col7/21(real_out11) -> fir_dbl_col8/21(real11)
  fir_dbl_col7/22(imag_out11) -> fir_dbl_col8/22(imag11)
  fir_dbl_col7/23(real_out12) -> fir_dbl_col8/23(real12)
  fir_dbl_col7/24(imag_out12) -> fir_dbl_col8/24(imag12)
  fir_dbl_col7/25(real_out13) -> fir_dbl_col8/25(real13)
  fir_dbl_col7/26(imag_out13) -> fir_dbl_col8/26(imag13)
  fir_dbl_col7/27(real_out14) -> fir_dbl_col8/27(real14)
  fir_dbl_col7/28(imag_out14) -> fir_dbl_col8/28(imag14)
  fir_dbl_col7/29(real_out15) -> fir_dbl_col8/29(real15)
  fir_dbl_col7/30(imag_out15) -> fir_dbl_col8/30(imag15)
  fir_dbl_col7/31(real_out16) -> fir_dbl_col8/31(real16)
  fir_dbl_col7/32(imag_out16) -> fir_dbl_col8/32(imag16)
  fir_dbl_col8/65(real_sum) -> real_sum/9(din8)
  fir_dbl_col8/66(imag_sum) -> imag_sum/9(din8)
  fir_dbl_col8/1(real_out1) -> fir_dbl_col9/1(real1)
  fir_dbl_col8/2(imag_out1) -> fir_dbl_col9/2(imag1)
  fir_dbl_col8/3(real_out2) -> fir_dbl_col9/3(real2)
  fir_dbl_col8/4(imag_out2) -> fir_dbl_col9/4(imag2)
  fir_dbl_col8/5(real_out3) -> fir_dbl_col9/5(real3)
  fir_dbl_col8/6(imag_out3) -> fir_dbl_col9/6(imag3)
  fir_dbl_col8/7(real_out4) -> fir_dbl_col9/7(real4)
  fir_dbl_col8/8(imag_out4) -> fir_dbl_col9/8(imag4)
  fir_dbl_col8/9(real_out5) -> fir_dbl_col9/9(real5)
  fir_dbl_col8/10(imag_out5) -> fir_dbl_col9/10(imag5)
  fir_dbl_col8/11(real_out6) -> fir_dbl_col9/11(real6)
  fir_dbl_col8/12(imag_out6) -> fir_dbl_col9/12(imag6)
  fir_dbl_col8/13(real_out7) -> fir_dbl_col9/13(real7)
  fir_dbl_col8/14(imag_out7) -> fir_dbl_col9/14(imag7)
  fir_dbl_col8/15(real_out8) -> fir_dbl_col9/15(real8)
  fir_dbl_col8/16(imag_out8) -> fir_dbl_col9/16(imag8)
  fir_dbl_col8/17(real_out9) -> fir_dbl_col9/17(real9)
  fir_dbl_col8/18(imag_out9) -> fir_dbl_col9/18(imag9)
  fir_dbl_col8/19(real_out10) -> fir_dbl_col9/19(real10)
  fir_dbl_col8/20(imag_out10) -> fir_dbl_col9/20(imag10)
  fir_dbl_col8/21(real_out11) -> fir_dbl_col9/21(real11)
  fir_dbl_col8/22(imag_out11) -> fir_dbl_col9/22(imag11)
  fir_dbl_col8/23(real_out12) -> fir_dbl_col9/23(real12)
  fir_dbl_col8/24(imag_out12) -> fir_dbl_col9/24(imag12)
  fir_dbl_col8/25(real_out13) -> fir_dbl_col9/25(real13)
  fir_dbl_col8/26(imag_out13) -> fir_dbl_col9/26(imag13)
  fir_dbl_col8/27(real_out14) -> fir_dbl_col9/27(real14)
  fir_dbl_col8/28(imag_out14) -> fir_dbl_col9/28(imag14)
  fir_dbl_col8/29(real_out15) -> fir_dbl_col9/29(real15)
  fir_dbl_col8/30(imag_out15) -> fir_dbl_col9/30(imag15)
  fir_dbl_col8/31(real_out16) -> fir_dbl_col9/31(real16)
  fir_dbl_col8/32(imag_out16) -> fir_dbl_col9/32(imag16)
  fir_dbl_col9/65(real_sum) -> real_sum/10(din9)
  fir_dbl_col9/66(imag_sum) -> imag_sum/10(din9)
  fir_dbl_col9/1(real_out1) -> fir_dbl_col10/1(real1)
  fir_dbl_col9/2(imag_out1) -> fir_dbl_col10/2(imag1)
  fir_dbl_col9/3(real_out2) -> fir_dbl_col10/3(real2)
  fir_dbl_col9/4(imag_out2) -> fir_dbl_col10/4(imag2)
  fir_dbl_col9/5(real_out3) -> fir_dbl_col10/5(real3)
  fir_dbl_col9/6(imag_out3) -> fir_dbl_col10/6(imag3)
  fir_dbl_col9/7(real_out4) -> fir_dbl_col10/7(real4)
  fir_dbl_col9/8(imag_out4) -> fir_dbl_col10/8(imag4)
  fir_dbl_col9/9(real_out5) -> fir_dbl_col10/9(real5)
  fir_dbl_col9/10(imag_out5) -> fir_dbl_col10/10(imag5)
  fir_dbl_col9/11(real_out6) -> fir_dbl_col10/11(real6)
  fir_dbl_col9/12(imag_out6) -> fir_dbl_col10/12(imag6)
  fir_dbl_col9/13(real_out7) -> fir_dbl_col10/13(real7)
  fir_dbl_col9/14(imag_out7) -> fir_dbl_col10/14(imag7)
  fir_dbl_col9/15(real_out8) -> fir_dbl_col10/15(real8)
  fir_dbl_col9/16(imag_out8) -> fir_dbl_col10/16(imag8)
  fir_dbl_col9/17(real_out9) -> fir_dbl_col10/17(real9)
  fir_dbl_col9/18(imag_out9) -> fir_dbl_col10/18(imag9)
  fir_dbl_col9/19(real_out10) -> fir_dbl_col10/19(real10)
  fir_dbl_col9/20(imag_out10) -> fir_dbl_col10/20(imag10)
  fir_dbl_col9/21(real_out11) -> fir_dbl_col10/21(real11)
  fir_dbl_col9/22(imag_out11) -> fir_dbl_col10/22(imag11)
  fir_dbl_col9/23(real_out12) -> fir_dbl_col10/23(real12)
  fir_dbl_col9/24(imag_out12) -> fir_dbl_col10/24(imag12)
  fir_dbl_col9/25(real_out13) -> fir_dbl_col10/25(real13)
  fir_dbl_col9/26(imag_out13) -> fir_dbl_col10/26(imag13)
  fir_dbl_col9/27(real_out14) -> fir_dbl_col10/27(real14)
  fir_dbl_col9/28(imag_out14) -> fir_dbl_col10/28(imag14)
  fir_dbl_col9/29(real_out15) -> fir_dbl_col10/29(real15)
  fir_dbl_col9/30(imag_out15) -> fir_dbl_col10/30(imag15)
  fir_dbl_col9/31(real_out16) -> fir_dbl_col10/31(real16)
  fir_dbl_col9/32(imag_out16) -> fir_dbl_col10/32(imag16)
  fir_dbl_col10/65(real_sum) -> real_sum/11(din10)
  fir_dbl_col10/66(imag_sum) -> imag_sum/11(din10)
  fir_dbl_col10/1(real_out1) -> fir_dbl_col11/1(real1)
  fir_dbl_col10/2(imag_out1) -> fir_dbl_col11/2(imag1)
  fir_dbl_col10/3(real_out2) -> fir_dbl_col11/3(real2)
  fir_dbl_col10/4(imag_out2) -> fir_dbl_col11/4(imag2)
  fir_dbl_col10/5(real_out3) -> fir_dbl_col11/5(real3)
  fir_dbl_col10/6(imag_out3) -> fir_dbl_col11/6(imag3)
  fir_dbl_col10/7(real_out4) -> fir_dbl_col11/7(real4)
  fir_dbl_col10/8(imag_out4) -> fir_dbl_col11/8(imag4)
  fir_dbl_col10/9(real_out5) -> fir_dbl_col11/9(real5)
  fir_dbl_col10/10(imag_out5) -> fir_dbl_col11/10(imag5)
  fir_dbl_col10/11(real_out6) -> fir_dbl_col11/11(real6)
  fir_dbl_col10/12(imag_out6) -> fir_dbl_col11/12(imag6)
  fir_dbl_col10/13(real_out7) -> fir_dbl_col11/13(real7)
  fir_dbl_col10/14(imag_out7) -> fir_dbl_col11/14(imag7)
  fir_dbl_col10/15(real_out8) -> fir_dbl_col11/15(real8)
  fir_dbl_col10/16(imag_out8) -> fir_dbl_col11/16(imag8)
  fir_dbl_col10/17(real_out9) -> fir_dbl_col11/17(real9)
  fir_dbl_col10/18(imag_out9) -> fir_dbl_col11/18(imag9)
  fir_dbl_col10/19(real_out10) -> fir_dbl_col11/19(real10)
  fir_dbl_col10/20(imag_out10) -> fir_dbl_col11/20(imag10)
  fir_dbl_col10/21(real_out11) -> fir_dbl_col11/21(real11)
  fir_dbl_col10/22(imag_out11) -> fir_dbl_col11/22(imag11)
  fir_dbl_col10/23(real_out12) -> fir_dbl_col11/23(real12)
  fir_dbl_col10/24(imag_out12) -> fir_dbl_col11/24(imag12)
  fir_dbl_col10/25(real_out13) -> fir_dbl_col11/25(real13)
  fir_dbl_col10/26(imag_out13) -> fir_dbl_col11/26(imag13)
  fir_dbl_col10/27(real_out14) -> fir_dbl_col11/27(real14)
  fir_dbl_col10/28(imag_out14) -> fir_dbl_col11/28(imag14)
  fir_dbl_col10/29(real_out15) -> fir_dbl_col11/29(real15)
  fir_dbl_col10/30(imag_out15) -> fir_dbl_col11/30(imag15)
  fir_dbl_col10/31(real_out16) -> fir_dbl_col11/31(real16)
  fir_dbl_col10/32(imag_out16) -> fir_dbl_col11/32(imag16)
  fir_dbl_col11/65(real_sum) -> real_sum/12(din11)
  fir_dbl_col11/66(imag_sum) -> imag_sum/12(din11)
  fir_dbl_col11/1(real_out1) -> fir_dbl_col12/1(real1)
  fir_dbl_col11/2(imag_out1) -> fir_dbl_col12/2(imag1)
  fir_dbl_col11/3(real_out2) -> fir_dbl_col12/3(real2)
  fir_dbl_col11/4(imag_out2) -> fir_dbl_col12/4(imag2)
  fir_dbl_col11/5(real_out3) -> fir_dbl_col12/5(real3)
  fir_dbl_col11/6(imag_out3) -> fir_dbl_col12/6(imag3)
  fir_dbl_col11/7(real_out4) -> fir_dbl_col12/7(real4)
  fir_dbl_col11/8(imag_out4) -> fir_dbl_col12/8(imag4)
  fir_dbl_col11/9(real_out5) -> fir_dbl_col12/9(real5)
  fir_dbl_col11/10(imag_out5) -> fir_dbl_col12/10(imag5)
  fir_dbl_col11/11(real_out6) -> fir_dbl_col12/11(real6)
  fir_dbl_col11/12(imag_out6) -> fir_dbl_col12/12(imag6)
  fir_dbl_col11/13(real_out7) -> fir_dbl_col12/13(real7)
  fir_dbl_col11/14(imag_out7) -> fir_dbl_col12/14(imag7)
  fir_dbl_col11/15(real_out8) -> fir_dbl_col12/15(real8)
  fir_dbl_col11/16(imag_out8) -> fir_dbl_col12/16(imag8)
  fir_dbl_col11/17(real_out9) -> fir_dbl_col12/17(real9)
  fir_dbl_col11/18(imag_out9) -> fir_dbl_col12/18(imag9)
  fir_dbl_col11/19(real_out10) -> fir_dbl_col12/19(real10)
  fir_dbl_col11/20(imag_out10) -> fir_dbl_col12/20(imag10)
  fir_dbl_col11/21(real_out11) -> fir_dbl_col12/21(real11)
  fir_dbl_col11/22(imag_out11) -> fir_dbl_col12/22(imag11)
  fir_dbl_col11/23(real_out12) -> fir_dbl_col12/23(real12)
  fir_dbl_col11/24(imag_out12) -> fir_dbl_col12/24(imag12)
  fir_dbl_col11/25(real_out13) -> fir_dbl_col12/25(real13)
  fir_dbl_col11/26(imag_out13) -> fir_dbl_col12/26(imag13)
  fir_dbl_col11/27(real_out14) -> fir_dbl_col12/27(real14)
  fir_dbl_col11/28(imag_out14) -> fir_dbl_col12/28(imag14)
  fir_dbl_col11/29(real_out15) -> fir_dbl_col12/29(real15)
  fir_dbl_col11/30(imag_out15) -> fir_dbl_col12/30(imag15)
  fir_dbl_col11/31(real_out16) -> fir_dbl_col12/31(real16)
  fir_dbl_col11/32(imag_out16) -> fir_dbl_col12/32(imag16)
  fir_dbl_col12/65(real_sum) -> real_sum/13(din12)
  fir_dbl_col12/66(imag_sum) -> imag_sum/13(din12)
  fir_dbl_col12/1(real_out1) -> fir_dbl_col13/1(real1)
  fir_dbl_col12/2(imag_out1) -> fir_dbl_col13/2(imag1)
  fir_dbl_col12/3(real_out2) -> fir_dbl_col13/3(real2)
  fir_dbl_col12/4(imag_out2) -> fir_dbl_col13/4(imag2)
  fir_dbl_col12/5(real_out3) -> fir_dbl_col13/5(real3)
  fir_dbl_col12/6(imag_out3) -> fir_dbl_col13/6(imag3)
  fir_dbl_col12/7(real_out4) -> fir_dbl_col13/7(real4)
  fir_dbl_col12/8(imag_out4) -> fir_dbl_col13/8(imag4)
  fir_dbl_col12/9(real_out5) -> fir_dbl_col13/9(real5)
  fir_dbl_col12/10(imag_out5) -> fir_dbl_col13/10(imag5)
  fir_dbl_col12/11(real_out6) -> fir_dbl_col13/11(real6)
  fir_dbl_col12/12(imag_out6) -> fir_dbl_col13/12(imag6)
  fir_dbl_col12/13(real_out7) -> fir_dbl_col13/13(real7)
  fir_dbl_col12/14(imag_out7) -> fir_dbl_col13/14(imag7)
  fir_dbl_col12/15(real_out8) -> fir_dbl_col13/15(real8)
  fir_dbl_col12/16(imag_out8) -> fir_dbl_col13/16(imag8)
  fir_dbl_col12/17(real_out9) -> fir_dbl_col13/17(real9)
  fir_dbl_col12/18(imag_out9) -> fir_dbl_col13/18(imag9)
  fir_dbl_col12/19(real_out10) -> fir_dbl_col13/19(real10)
  fir_dbl_col12/20(imag_out10) -> fir_dbl_col13/20(imag10)
  fir_dbl_col12/21(real_out11) -> fir_dbl_col13/21(real11)
  fir_dbl_col12/22(imag_out11) -> fir_dbl_col13/22(imag11)
  fir_dbl_col12/23(real_out12) -> fir_dbl_col13/23(real12)
  fir_dbl_col12/24(imag_out12) -> fir_dbl_col13/24(imag12)
  fir_dbl_col12/25(real_out13) -> fir_dbl_col13/25(real13)
  fir_dbl_col12/26(imag_out13) -> fir_dbl_col13/26(imag13)
  fir_dbl_col12/27(real_out14) -> fir_dbl_col13/27(real14)
  fir_dbl_col12/28(imag_out14) -> fir_dbl_col13/28(imag14)
  fir_dbl_col12/29(real_out15) -> fir_dbl_col13/29(real15)
  fir_dbl_col12/30(imag_out15) -> fir_dbl_col13/30(imag15)
  fir_dbl_col12/31(real_out16) -> fir_dbl_col13/31(real16)
  fir_dbl_col12/32(imag_out16) -> fir_dbl_col13/32(imag16)
  fir_dbl_col13/65(real_sum) -> real_sum/14(din13)
  fir_dbl_col13/66(imag_sum) -> imag_sum/14(din13)
  fir_dbl_col13/1(real_out1) -> fir_dbl_col14/1(real1)
  fir_dbl_col13/2(imag_out1) -> fir_dbl_col14/2(imag1)
  fir_dbl_col13/3(real_out2) -> fir_dbl_col14/3(real2)
  fir_dbl_col13/4(imag_out2) -> fir_dbl_col14/4(imag2)
  fir_dbl_col13/5(real_out3) -> fir_dbl_col14/5(real3)
  fir_dbl_col13/6(imag_out3) -> fir_dbl_col14/6(imag3)
  fir_dbl_col13/7(real_out4) -> fir_dbl_col14/7(real4)
  fir_dbl_col13/8(imag_out4) -> fir_dbl_col14/8(imag4)
  fir_dbl_col13/9(real_out5) -> fir_dbl_col14/9(real5)
  fir_dbl_col13/10(imag_out5) -> fir_dbl_col14/10(imag5)
  fir_dbl_col13/11(real_out6) -> fir_dbl_col14/11(real6)
  fir_dbl_col13/12(imag_out6) -> fir_dbl_col14/12(imag6)
  fir_dbl_col13/13(real_out7) -> fir_dbl_col14/13(real7)
  fir_dbl_col13/14(imag_out7) -> fir_dbl_col14/14(imag7)
  fir_dbl_col13/15(real_out8) -> fir_dbl_col14/15(real8)
  fir_dbl_col13/16(imag_out8) -> fir_dbl_col14/16(imag8)
  fir_dbl_col13/17(real_out9) -> fir_dbl_col14/17(real9)
  fir_dbl_col13/18(imag_out9) -> fir_dbl_col14/18(imag9)
  fir_dbl_col13/19(real_out10) -> fir_dbl_col14/19(real10)
  fir_dbl_col13/20(imag_out10) -> fir_dbl_col14/20(imag10)
  fir_dbl_col13/21(real_out11) -> fir_dbl_col14/21(real11)
  fir_dbl_col13/22(imag_out11) -> fir_dbl_col14/22(imag11)
  fir_dbl_col13/23(real_out12) -> fir_dbl_col14/23(real12)
  fir_dbl_col13/24(imag_out12) -> fir_dbl_col14/24(imag12)
  fir_dbl_col13/25(real_out13) -> fir_dbl_col14/25(real13)
  fir_dbl_col13/26(imag_out13) -> fir_dbl_col14/26(imag13)
  fir_dbl_col13/27(real_out14) -> fir_dbl_col14/27(real14)
  fir_dbl_col13/28(imag_out14) -> fir_dbl_col14/28(imag14)
  fir_dbl_col13/29(real_out15) -> fir_dbl_col14/29(real15)
  fir_dbl_col13/30(imag_out15) -> fir_dbl_col14/30(imag15)
  fir_dbl_col13/31(real_out16) -> fir_dbl_col14/31(real16)
  fir_dbl_col13/32(imag_out16) -> fir_dbl_col14/32(imag16)
  fir_dbl_col14/65(real_sum) -> real_sum/15(din14)
  fir_dbl_col14/66(imag_sum) -> imag_sum/15(din14)
  fir_dbl_col14/1(real_out1) -> fir_dbl_col15/1(real1)
  fir_dbl_col14/2(imag_out1) -> fir_dbl_col15/2(imag1)
  fir_dbl_col14/3(real_out2) -> fir_dbl_col15/3(real2)
  fir_dbl_col14/4(imag_out2) -> fir_dbl_col15/4(imag2)
  fir_dbl_col14/5(real_out3) -> fir_dbl_col15/5(real3)
  fir_dbl_col14/6(imag_out3) -> fir_dbl_col15/6(imag3)
  fir_dbl_col14/7(real_out4) -> fir_dbl_col15/7(real4)
  fir_dbl_col14/8(imag_out4) -> fir_dbl_col15/8(imag4)
  fir_dbl_col14/9(real_out5) -> fir_dbl_col15/9(real5)
  fir_dbl_col14/10(imag_out5) -> fir_dbl_col15/10(imag5)
  fir_dbl_col14/11(real_out6) -> fir_dbl_col15/11(real6)
  fir_dbl_col14/12(imag_out6) -> fir_dbl_col15/12(imag6)
  fir_dbl_col14/13(real_out7) -> fir_dbl_col15/13(real7)
  fir_dbl_col14/14(imag_out7) -> fir_dbl_col15/14(imag7)
  fir_dbl_col14/15(real_out8) -> fir_dbl_col15/15(real8)
  fir_dbl_col14/16(imag_out8) -> fir_dbl_col15/16(imag8)
  fir_dbl_col14/17(real_out9) -> fir_dbl_col15/17(real9)
  fir_dbl_col14/18(imag_out9) -> fir_dbl_col15/18(imag9)
  fir_dbl_col14/19(real_out10) -> fir_dbl_col15/19(real10)
  fir_dbl_col14/20(imag_out10) -> fir_dbl_col15/20(imag10)
  fir_dbl_col14/21(real_out11) -> fir_dbl_col15/21(real11)
  fir_dbl_col14/22(imag_out11) -> fir_dbl_col15/22(imag11)
  fir_dbl_col14/23(real_out12) -> fir_dbl_col15/23(real12)
  fir_dbl_col14/24(imag_out12) -> fir_dbl_col15/24(imag12)
  fir_dbl_col14/25(real_out13) -> fir_dbl_col15/25(real13)
  fir_dbl_col14/26(imag_out13) -> fir_dbl_col15/26(imag13)
  fir_dbl_col14/27(real_out14) -> fir_dbl_col15/27(real14)
  fir_dbl_col14/28(imag_out14) -> fir_dbl_col15/28(imag14)
  fir_dbl_col14/29(real_out15) -> fir_dbl_col15/29(real15)
  fir_dbl_col14/30(imag_out15) -> fir_dbl_col15/30(imag15)
  fir_dbl_col14/31(real_out16) -> fir_dbl_col15/31(real16)
  fir_dbl_col14/32(imag_out16) -> fir_dbl_col15/32(imag16)
  fir_dbl_col15/65(real_sum) -> real_sum/16(din15)
  fir_dbl_col15/66(imag_sum) -> imag_sum/16(din15)
  fir_dbl_col15/1(real_out1) -> fir_dbl_col16/1(real1)
  fir_dbl_col15/2(imag_out1) -> fir_dbl_col16/2(imag1)
  fir_dbl_col15/3(real_out2) -> fir_dbl_col16/3(real2)
  fir_dbl_col15/4(imag_out2) -> fir_dbl_col16/4(imag2)
  fir_dbl_col15/5(real_out3) -> fir_dbl_col16/5(real3)
  fir_dbl_col15/6(imag_out3) -> fir_dbl_col16/6(imag3)
  fir_dbl_col15/7(real_out4) -> fir_dbl_col16/7(real4)
  fir_dbl_col15/8(imag_out4) -> fir_dbl_col16/8(imag4)
  fir_dbl_col15/9(real_out5) -> fir_dbl_col16/9(real5)
  fir_dbl_col15/10(imag_out5) -> fir_dbl_col16/10(imag5)
  fir_dbl_col15/11(real_out6) -> fir_dbl_col16/11(real6)
  fir_dbl_col15/12(imag_out6) -> fir_dbl_col16/12(imag6)
  fir_dbl_col15/13(real_out7) -> fir_dbl_col16/13(real7)
  fir_dbl_col15/14(imag_out7) -> fir_dbl_col16/14(imag7)
  fir_dbl_col15/15(real_out8) -> fir_dbl_col16/15(real8)
  fir_dbl_col15/16(imag_out8) -> fir_dbl_col16/16(imag8)
  fir_dbl_col15/17(real_out9) -> fir_dbl_col16/17(real9)
  fir_dbl_col15/18(imag_out9) -> fir_dbl_col16/18(imag9)
  fir_dbl_col15/19(real_out10) -> fir_dbl_col16/19(real10)
  fir_dbl_col15/20(imag_out10) -> fir_dbl_col16/20(imag10)
  fir_dbl_col15/21(real_out11) -> fir_dbl_col16/21(real11)
  fir_dbl_col15/22(imag_out11) -> fir_dbl_col16/22(imag11)
  fir_dbl_col15/23(real_out12) -> fir_dbl_col16/23(real12)
  fir_dbl_col15/24(imag_out12) -> fir_dbl_col16/24(imag12)
  fir_dbl_col15/25(real_out13) -> fir_dbl_col16/25(real13)
  fir_dbl_col15/26(imag_out13) -> fir_dbl_col16/26(imag13)
  fir_dbl_col15/27(real_out14) -> fir_dbl_col16/27(real14)
  fir_dbl_col15/28(imag_out14) -> fir_dbl_col16/28(imag14)
  fir_dbl_col15/29(real_out15) -> fir_dbl_col16/29(real15)
  fir_dbl_col15/30(imag_out15) -> fir_dbl_col16/30(imag15)
  fir_dbl_col15/31(real_out16) -> fir_dbl_col16/31(real16)
  fir_dbl_col15/32(imag_out16) -> fir_dbl_col16/32(imag16)
  fir_dbl_col16/65(real_sum) -> real_sum/17(din16)
  fir_dbl_col16/66(imag_sum) -> imag_sum/17(din16)
  real_sum/2(dout) -> shift1/1
  imag_sum/2(dout) -> shift2/1
  shift1/1 -> convert1/1
  shift2/1 -> convert2/1
  convert1/1 -> ri_to_c/1
  convert2/1 -> ri_to_c/2
  ri_to_c/1 -> dout/1
  sync_in/1 -> delay/1
  delay/1 -> real_sum/1(sync), imag_sum/1(sync)
  real_sum/1(sync_out) -> sync_out/1
  fir_dbl_col2/33(real_back_out1) -> fir_dbl_col1/33(real_back1)
  fir_dbl_col2/34(imag_back_out1) -> fir_dbl_col1/34(imag_back1)
  fir_dbl_col2/35(real_back_out2) -> fir_dbl_col1/35(real_back2)
  fir_dbl_col2/36(imag_back_out2) -> fir_dbl_col1/36(imag_back2)
  fir_dbl_col2/37(real_back_out3) -> fir_dbl_col1/37(real_back3)
  fir_dbl_col2/38(imag_back_out3) -> fir_dbl_col1/38(imag_back3)
  fir_dbl_col2/39(real_back_out4) -> fir_dbl_col1/39(real_back4)
  fir_dbl_col2/40(imag_back_out4) -> fir_dbl_col1/40(imag_back4)
  fir_dbl_col2/41(real_back_out5) -> fir_dbl_col1/41(real_back5)
  fir_dbl_col2/42(imag_back_out5) -> fir_dbl_col1/42(imag_back5)
  fir_dbl_col2/43(real_back_out6) -> fir_dbl_col1/43(real_back6)
  fir_dbl_col2/44(imag_back_out6) -> fir_dbl_col1/44(imag_back6)
  fir_dbl_col2/45(real_back_out7) -> fir_dbl_col1/45(real_back7)
  fir_dbl_col2/46(imag_back_out7) -> fir_dbl_col1/46(imag_back7)
  fir_dbl_col2/47(real_back_out8) -> fir_dbl_col1/47(real_back8)
  fir_dbl_col2/48(imag_back_out8) -> fir_dbl_col1/48(imag_back8)
  fir_dbl_col2/49(real_back_out9) -> fir_dbl_col1/49(real_back9)
  fir_dbl_col2/50(imag_back_out9) -> fir_dbl_col1/50(imag_back9)
  fir_dbl_col2/51(real_back_out10) -> fir_dbl_col1/51(real_back10)
  fir_dbl_col2/52(imag_back_out10) -> fir_dbl_col1/52(imag_back10)
  fir_dbl_col2/53(real_back_out11) -> fir_dbl_col1/53(real_back11)
  fir_dbl_col2/54(imag_back_out11) -> fir_dbl_col1/54(imag_back11)
  fir_dbl_col2/55(real_back_out12) -> fir_dbl_col1/55(real_back12)
  fir_dbl_col2/56(imag_back_out12) -> fir_dbl_col1/56(imag_back12)
  fir_dbl_col2/57(real_back_out13) -> fir_dbl_col1/57(real_back13)
  fir_dbl_col2/58(imag_back_out13) -> fir_dbl_col1/58(imag_back13)
  fir_dbl_col2/59(real_back_out14) -> fir_dbl_col1/59(real_back14)
  fir_dbl_col2/60(imag_back_out14) -> fir_dbl_col1/60(imag_back14)
  fir_dbl_col2/61(real_back_out15) -> fir_dbl_col1/61(real_back15)
  fir_dbl_col2/62(imag_back_out15) -> fir_dbl_col1/62(imag_back15)
  fir_dbl_col2/63(real_back_out16) -> fir_dbl_col1/63(real_back16)
  fir_dbl_col2/64(imag_back_out16) -> fir_dbl_col1/64(imag_back16)
  fir_dbl_col3/33(real_back_out1) -> fir_dbl_col2/33(real_back1)
  fir_dbl_col3/34(imag_back_out1) -> fir_dbl_col2/34(imag_back1)
  fir_dbl_col3/35(real_back_out2) -> fir_dbl_col2/35(real_back2)
  fir_dbl_col3/36(imag_back_out2) -> fir_dbl_col2/36(imag_back2)
  fir_dbl_col3/37(real_back_out3) -> fir_dbl_col2/37(real_back3)
  fir_dbl_col3/38(imag_back_out3) -> fir_dbl_col2/38(imag_back3)
  fir_dbl_col3/39(real_back_out4) -> fir_dbl_col2/39(real_back4)
  fir_dbl_col3/40(imag_back_out4) -> fir_dbl_col2/40(imag_back4)
  fir_dbl_col3/41(real_back_out5) -> fir_dbl_col2/41(real_back5)
  fir_dbl_col3/42(imag_back_out5) -> fir_dbl_col2/42(imag_back5)
  fir_dbl_col3/43(real_back_out6) -> fir_dbl_col2/43(real_back6)
  fir_dbl_col3/44(imag_back_out6) -> fir_dbl_col2/44(imag_back6)
  fir_dbl_col3/45(real_back_out7) -> fir_dbl_col2/45(real_back7)
  fir_dbl_col3/46(imag_back_out7) -> fir_dbl_col2/46(imag_back7)
  fir_dbl_col3/47(real_back_out8) -> fir_dbl_col2/47(real_back8)
  fir_dbl_col3/48(imag_back_out8) -> fir_dbl_col2/48(imag_back8)
  fir_dbl_col3/49(real_back_out9) -> fir_dbl_col2/49(real_back9)
  fir_dbl_col3/50(imag_back_out9) -> fir_dbl_col2/50(imag_back9)
  fir_dbl_col3/51(real_back_out10) -> fir_dbl_col2/51(real_back10)
  fir_dbl_col3/52(imag_back_out10) -> fir_dbl_col2/52(imag_back10)
  fir_dbl_col3/53(real_back_out11) -> fir_dbl_col2/53(real_back11)
  fir_dbl_col3/54(imag_back_out11) -> fir_dbl_col2/54(imag_back11)
  fir_dbl_col3/55(real_back_out12) -> fir_dbl_col2/55(real_back12)
  fir_dbl_col3/56(imag_back_out12) -> fir_dbl_col2/56(imag_back12)
  fir_dbl_col3/57(real_back_out13) -> fir_dbl_col2/57(real_back13)
  fir_dbl_col3/58(imag_back_out13) -> fir_dbl_col2/58(imag_back13)
  fir_dbl_col3/59(real_back_out14) -> fir_dbl_col2/59(real_back14)
  fir_dbl_col3/60(imag_back_out14) -> fir_dbl_col2/60(imag_back14)
  fir_dbl_col3/61(real_back_out15) -> fir_dbl_col2/61(real_back15)
  fir_dbl_col3/62(imag_back_out15) -> fir_dbl_col2/62(imag_back15)
  fir_dbl_col3/63(real_back_out16) -> fir_dbl_col2/63(real_back16)
  fir_dbl_col3/64(imag_back_out16) -> fir_dbl_col2/64(imag_back16)
  fir_dbl_col4/33(real_back_out1) -> fir_dbl_col3/33(real_back1)
  fir_dbl_col4/34(imag_back_out1) -> fir_dbl_col3/34(imag_back1)
  fir_dbl_col4/35(real_back_out2) -> fir_dbl_col3/35(real_back2)
  fir_dbl_col4/36(imag_back_out2) -> fir_dbl_col3/36(imag_back2)
  fir_dbl_col4/37(real_back_out3) -> fir_dbl_col3/37(real_back3)
  fir_dbl_col4/38(imag_back_out3) -> fir_dbl_col3/38(imag_back3)
  fir_dbl_col4/39(real_back_out4) -> fir_dbl_col3/39(real_back4)
  fir_dbl_col4/40(imag_back_out4) -> fir_dbl_col3/40(imag_back4)
  fir_dbl_col4/41(real_back_out5) -> fir_dbl_col3/41(real_back5)
  fir_dbl_col4/42(imag_back_out5) -> fir_dbl_col3/42(imag_back5)
  fir_dbl_col4/43(real_back_out6) -> fir_dbl_col3/43(real_back6)
  fir_dbl_col4/44(imag_back_out6) -> fir_dbl_col3/44(imag_back6)
  fir_dbl_col4/45(real_back_out7) -> fir_dbl_col3/45(real_back7)
  fir_dbl_col4/46(imag_back_out7) -> fir_dbl_col3/46(imag_back7)
  fir_dbl_col4/47(real_back_out8) -> fir_dbl_col3/47(real_back8)
  fir_dbl_col4/48(imag_back_out8) -> fir_dbl_col3/48(imag_back8)
  fir_dbl_col4/49(real_back_out9) -> fir_dbl_col3/49(real_back9)
  fir_dbl_col4/50(imag_back_out9) -> fir_dbl_col3/50(imag_back9)
  fir_dbl_col4/51(real_back_out10) -> fir_dbl_col3/51(real_back10)
  fir_dbl_col4/52(imag_back_out10) -> fir_dbl_col3/52(imag_back10)
  fir_dbl_col4/53(real_back_out11) -> fir_dbl_col3/53(real_back11)
  fir_dbl_col4/54(imag_back_out11) -> fir_dbl_col3/54(imag_back11)
  fir_dbl_col4/55(real_back_out12) -> fir_dbl_col3/55(real_back12)
  fir_dbl_col4/56(imag_back_out12) -> fir_dbl_col3/56(imag_back12)
  fir_dbl_col4/57(real_back_out13) -> fir_dbl_col3/57(real_back13)
  fir_dbl_col4/58(imag_back_out13) -> fir_dbl_col3/58(imag_back13)
  fir_dbl_col4/59(real_back_out14) -> fir_dbl_col3/59(real_back14)
  fir_dbl_col4/60(imag_back_out14) -> fir_dbl_col3/60(imag_back14)
  fir_dbl_col4/61(real_back_out15) -> fir_dbl_col3/61(real_back15)
  fir_dbl_col4/62(imag_back_out15) -> fir_dbl_col3/62(imag_back15)
  fir_dbl_col4/63(real_back_out16) -> fir_dbl_col3/63(real_back16)
  fir_dbl_col4/64(imag_back_out16) -> fir_dbl_col3/64(imag_back16)
  fir_dbl_col5/33(real_back_out1) -> fir_dbl_col4/33(real_back1)
  fir_dbl_col5/34(imag_back_out1) -> fir_dbl_col4/34(imag_back1)
  fir_dbl_col5/35(real_back_out2) -> fir_dbl_col4/35(real_back2)
  fir_dbl_col5/36(imag_back_out2) -> fir_dbl_col4/36(imag_back2)
  fir_dbl_col5/37(real_back_out3) -> fir_dbl_col4/37(real_back3)
  fir_dbl_col5/38(imag_back_out3) -> fir_dbl_col4/38(imag_back3)
  fir_dbl_col5/39(real_back_out4) -> fir_dbl_col4/39(real_back4)
  fir_dbl_col5/40(imag_back_out4) -> fir_dbl_col4/40(imag_back4)
  fir_dbl_col5/41(real_back_out5) -> fir_dbl_col4/41(real_back5)
  fir_dbl_col5/42(imag_back_out5) -> fir_dbl_col4/42(imag_back5)
  fir_dbl_col5/43(real_back_out6) -> fir_dbl_col4/43(real_back6)
  fir_dbl_col5/44(imag_back_out6) -> fir_dbl_col4/44(imag_back6)
  fir_dbl_col5/45(real_back_out7) -> fir_dbl_col4/45(real_back7)
  fir_dbl_col5/46(imag_back_out7) -> fir_dbl_col4/46(imag_back7)
  fir_dbl_col5/47(real_back_out8) -> fir_dbl_col4/47(real_back8)
  fir_dbl_col5/48(imag_back_out8) -> fir_dbl_col4/48(imag_back8)
  fir_dbl_col5/49(real_back_out9) -> fir_dbl_col4/49(real_back9)
  fir_dbl_col5/50(imag_back_out9) -> fir_dbl_col4/50(imag_back9)
  fir_dbl_col5/51(real_back_out10) -> fir_dbl_col4/51(real_back10)
  fir_dbl_col5/52(imag_back_out10) -> fir_dbl_col4/52(imag_back10)
  fir_dbl_col5/53(real_back_out11) -> fir_dbl_col4/53(real_back11)
  fir_dbl_col5/54(imag_back_out11) -> fir_dbl_col4/54(imag_back11)
  fir_dbl_col5/55(real_back_out12) -> fir_dbl_col4/55(real_back12)
  fir_dbl_col5/56(imag_back_out12) -> fir_dbl_col4/56(imag_back12)
  fir_dbl_col5/57(real_back_out13) -> fir_dbl_col4/57(real_back13)
  fir_dbl_col5/58(imag_back_out13) -> fir_dbl_col4/58(imag_back13)
  fir_dbl_col5/59(real_back_out14) -> fir_dbl_col4/59(real_back14)
  fir_dbl_col5/60(imag_back_out14) -> fir_dbl_col4/60(imag_back14)
  fir_dbl_col5/61(real_back_out15) -> fir_dbl_col4/61(real_back15)
  fir_dbl_col5/62(imag_back_out15) -> fir_dbl_col4/62(imag_back15)
  fir_dbl_col5/63(real_back_out16) -> fir_dbl_col4/63(real_back16)
  fir_dbl_col5/64(imag_back_out16) -> fir_dbl_col4/64(imag_back16)
  fir_dbl_col6/33(real_back_out1) -> fir_dbl_col5/33(real_back1)
  fir_dbl_col6/34(imag_back_out1) -> fir_dbl_col5/34(imag_back1)
  fir_dbl_col6/35(real_back_out2) -> fir_dbl_col5/35(real_back2)
  fir_dbl_col6/36(imag_back_out2) -> fir_dbl_col5/36(imag_back2)
  fir_dbl_col6/37(real_back_out3) -> fir_dbl_col5/37(real_back3)
  fir_dbl_col6/38(imag_back_out3) -> fir_dbl_col5/38(imag_back3)
  fir_dbl_col6/39(real_back_out4) -> fir_dbl_col5/39(real_back4)
  fir_dbl_col6/40(imag_back_out4) -> fir_dbl_col5/40(imag_back4)
  fir_dbl_col6/41(real_back_out5) -> fir_dbl_col5/41(real_back5)
  fir_dbl_col6/42(imag_back_out5) -> fir_dbl_col5/42(imag_back5)
  fir_dbl_col6/43(real_back_out6) -> fir_dbl_col5/43(real_back6)
  fir_dbl_col6/44(imag_back_out6) -> fir_dbl_col5/44(imag_back6)
  fir_dbl_col6/45(real_back_out7) -> fir_dbl_col5/45(real_back7)
  fir_dbl_col6/46(imag_back_out7) -> fir_dbl_col5/46(imag_back7)
  fir_dbl_col6/47(real_back_out8) -> fir_dbl_col5/47(real_back8)
  fir_dbl_col6/48(imag_back_out8) -> fir_dbl_col5/48(imag_back8)
  fir_dbl_col6/49(real_back_out9) -> fir_dbl_col5/49(real_back9)
  fir_dbl_col6/50(imag_back_out9) -> fir_dbl_col5/50(imag_back9)
  fir_dbl_col6/51(real_back_out10) -> fir_dbl_col5/51(real_back10)
  fir_dbl_col6/52(imag_back_out10) -> fir_dbl_col5/52(imag_back10)
  fir_dbl_col6/53(real_back_out11) -> fir_dbl_col5/53(real_back11)
  fir_dbl_col6/54(imag_back_out11) -> fir_dbl_col5/54(imag_back11)
  fir_dbl_col6/55(real_back_out12) -> fir_dbl_col5/55(real_back12)
  fir_dbl_col6/56(imag_back_out12) -> fir_dbl_col5/56(imag_back12)
  fir_dbl_col6/57(real_back_out13) -> fir_dbl_col5/57(real_back13)
  fir_dbl_col6/58(imag_back_out13) -> fir_dbl_col5/58(imag_back13)
  fir_dbl_col6/59(real_back_out14) -> fir_dbl_col5/59(real_back14)
  fir_dbl_col6/60(imag_back_out14) -> fir_dbl_col5/60(imag_back14)
  fir_dbl_col6/61(real_back_out15) -> fir_dbl_col5/61(real_back15)
  fir_dbl_col6/62(imag_back_out15) -> fir_dbl_col5/62(imag_back15)
  fir_dbl_col6/63(real_back_out16) -> fir_dbl_col5/63(real_back16)
  fir_dbl_col6/64(imag_back_out16) -> fir_dbl_col5/64(imag_back16)
  fir_dbl_col7/33(real_back_out1) -> fir_dbl_col6/33(real_back1)
  fir_dbl_col7/34(imag_back_out1) -> fir_dbl_col6/34(imag_back1)
  fir_dbl_col7/35(real_back_out2) -> fir_dbl_col6/35(real_back2)
  fir_dbl_col7/36(imag_back_out2) -> fir_dbl_col6/36(imag_back2)
  fir_dbl_col7/37(real_back_out3) -> fir_dbl_col6/37(real_back3)
  fir_dbl_col7/38(imag_back_out3) -> fir_dbl_col6/38(imag_back3)
  fir_dbl_col7/39(real_back_out4) -> fir_dbl_col6/39(real_back4)
  fir_dbl_col7/40(imag_back_out4) -> fir_dbl_col6/40(imag_back4)
  fir_dbl_col7/41(real_back_out5) -> fir_dbl_col6/41(real_back5)
  fir_dbl_col7/42(imag_back_out5) -> fir_dbl_col6/42(imag_back5)
  fir_dbl_col7/43(real_back_out6) -> fir_dbl_col6/43(real_back6)
  fir_dbl_col7/44(imag_back_out6) -> fir_dbl_col6/44(imag_back6)
  fir_dbl_col7/45(real_back_out7) -> fir_dbl_col6/45(real_back7)
  fir_dbl_col7/46(imag_back_out7) -> fir_dbl_col6/46(imag_back7)
  fir_dbl_col7/47(real_back_out8) -> fir_dbl_col6/47(real_back8)
  fir_dbl_col7/48(imag_back_out8) -> fir_dbl_col6/48(imag_back8)
  fir_dbl_col7/49(real_back_out9) -> fir_dbl_col6/49(real_back9)
  fir_dbl_col7/50(imag_back_out9) -> fir_dbl_col6/50(imag_back9)
  fir_dbl_col7/51(real_back_out10) -> fir_dbl_col6/51(real_back10)
  fir_dbl_col7/52(imag_back_out10) -> fir_dbl_col6/52(imag_back10)
  fir_dbl_col7/53(real_back_out11) -> fir_dbl_col6/53(real_back11)
  fir_dbl_col7/54(imag_back_out11) -> fir_dbl_col6/54(imag_back11)
  fir_dbl_col7/55(real_back_out12) -> fir_dbl_col6/55(real_back12)
  fir_dbl_col7/56(imag_back_out12) -> fir_dbl_col6/56(imag_back12)
  fir_dbl_col7/57(real_back_out13) -> fir_dbl_col6/57(real_back13)
  fir_dbl_col7/58(imag_back_out13) -> fir_dbl_col6/58(imag_back13)
  fir_dbl_col7/59(real_back_out14) -> fir_dbl_col6/59(real_back14)
  fir_dbl_col7/60(imag_back_out14) -> fir_dbl_col6/60(imag_back14)
  fir_dbl_col7/61(real_back_out15) -> fir_dbl_col6/61(real_back15)
  fir_dbl_col7/62(imag_back_out15) -> fir_dbl_col6/62(imag_back15)
  fir_dbl_col7/63(real_back_out16) -> fir_dbl_col6/63(real_back16)
  fir_dbl_col7/64(imag_back_out16) -> fir_dbl_col6/64(imag_back16)
  fir_dbl_col8/33(real_back_out1) -> fir_dbl_col7/33(real_back1)
  fir_dbl_col8/34(imag_back_out1) -> fir_dbl_col7/34(imag_back1)
  fir_dbl_col8/35(real_back_out2) -> fir_dbl_col7/35(real_back2)
  fir_dbl_col8/36(imag_back_out2) -> fir_dbl_col7/36(imag_back2)
  fir_dbl_col8/37(real_back_out3) -> fir_dbl_col7/37(real_back3)
  fir_dbl_col8/38(imag_back_out3) -> fir_dbl_col7/38(imag_back3)
  fir_dbl_col8/39(real_back_out4) -> fir_dbl_col7/39(real_back4)
  fir_dbl_col8/40(imag_back_out4) -> fir_dbl_col7/40(imag_back4)
  fir_dbl_col8/41(real_back_out5) -> fir_dbl_col7/41(real_back5)
  fir_dbl_col8/42(imag_back_out5) -> fir_dbl_col7/42(imag_back5)
  fir_dbl_col8/43(real_back_out6) -> fir_dbl_col7/43(real_back6)
  fir_dbl_col8/44(imag_back_out6) -> fir_dbl_col7/44(imag_back6)
  fir_dbl_col8/45(real_back_out7) -> fir_dbl_col7/45(real_back7)
  fir_dbl_col8/46(imag_back_out7) -> fir_dbl_col7/46(imag_back7)
  fir_dbl_col8/47(real_back_out8) -> fir_dbl_col7/47(real_back8)
  fir_dbl_col8/48(imag_back_out8) -> fir_dbl_col7/48(imag_back8)
  fir_dbl_col8/49(real_back_out9) -> fir_dbl_col7/49(real_back9)
  fir_dbl_col8/50(imag_back_out9) -> fir_dbl_col7/50(imag_back9)
  fir_dbl_col8/51(real_back_out10) -> fir_dbl_col7/51(real_back10)
  fir_dbl_col8/52(imag_back_out10) -> fir_dbl_col7/52(imag_back10)
  fir_dbl_col8/53(real_back_out11) -> fir_dbl_col7/53(real_back11)
  fir_dbl_col8/54(imag_back_out11) -> fir_dbl_col7/54(imag_back11)
  fir_dbl_col8/55(real_back_out12) -> fir_dbl_col7/55(real_back12)
  fir_dbl_col8/56(imag_back_out12) -> fir_dbl_col7/56(imag_back12)
  fir_dbl_col8/57(real_back_out13) -> fir_dbl_col7/57(real_back13)
  fir_dbl_col8/58(imag_back_out13) -> fir_dbl_col7/58(imag_back13)
  fir_dbl_col8/59(real_back_out14) -> fir_dbl_col7/59(real_back14)
  fir_dbl_col8/60(imag_back_out14) -> fir_dbl_col7/60(imag_back14)
  fir_dbl_col8/61(real_back_out15) -> fir_dbl_col7/61(real_back15)
  fir_dbl_col8/62(imag_back_out15) -> fir_dbl_col7/62(imag_back15)
  fir_dbl_col8/63(real_back_out16) -> fir_dbl_col7/63(real_back16)
  fir_dbl_col8/64(imag_back_out16) -> fir_dbl_col7/64(imag_back16)
  fir_dbl_col9/33(real_back_out1) -> fir_dbl_col8/33(real_back1)
  fir_dbl_col9/34(imag_back_out1) -> fir_dbl_col8/34(imag_back1)
  fir_dbl_col9/35(real_back_out2) -> fir_dbl_col8/35(real_back2)
  fir_dbl_col9/36(imag_back_out2) -> fir_dbl_col8/36(imag_back2)
  fir_dbl_col9/37(real_back_out3) -> fir_dbl_col8/37(real_back3)
  fir_dbl_col9/38(imag_back_out3) -> fir_dbl_col8/38(imag_back3)
  fir_dbl_col9/39(real_back_out4) -> fir_dbl_col8/39(real_back4)
  fir_dbl_col9/40(imag_back_out4) -> fir_dbl_col8/40(imag_back4)
  fir_dbl_col9/41(real_back_out5) -> fir_dbl_col8/41(real_back5)
  fir_dbl_col9/42(imag_back_out5) -> fir_dbl_col8/42(imag_back5)
  fir_dbl_col9/43(real_back_out6) -> fir_dbl_col8/43(real_back6)
  fir_dbl_col9/44(imag_back_out6) -> fir_dbl_col8/44(imag_back6)
  fir_dbl_col9/45(real_back_out7) -> fir_dbl_col8/45(real_back7)
  fir_dbl_col9/46(imag_back_out7) -> fir_dbl_col8/46(imag_back7)
  fir_dbl_col9/47(real_back_out8) -> fir_dbl_col8/47(real_back8)
  fir_dbl_col9/48(imag_back_out8) -> fir_dbl_col8/48(imag_back8)
  fir_dbl_col9/49(real_back_out9) -> fir_dbl_col8/49(real_back9)
  fir_dbl_col9/50(imag_back_out9) -> fir_dbl_col8/50(imag_back9)
  fir_dbl_col9/51(real_back_out10) -> fir_dbl_col8/51(real_back10)
  fir_dbl_col9/52(imag_back_out10) -> fir_dbl_col8/52(imag_back10)
  fir_dbl_col9/53(real_back_out11) -> fir_dbl_col8/53(real_back11)
  fir_dbl_col9/54(imag_back_out11) -> fir_dbl_col8/54(imag_back11)
  fir_dbl_col9/55(real_back_out12) -> fir_dbl_col8/55(real_back12)
  fir_dbl_col9/56(imag_back_out12) -> fir_dbl_col8/56(imag_back12)
  fir_dbl_col9/57(real_back_out13) -> fir_dbl_col8/57(real_back13)
  fir_dbl_col9/58(imag_back_out13) -> fir_dbl_col8/58(imag_back13)
  fir_dbl_col9/59(real_back_out14) -> fir_dbl_col8/59(real_back14)
  fir_dbl_col9/60(imag_back_out14) -> fir_dbl_col8/60(imag_back14)
  fir_dbl_col9/61(real_back_out15) -> fir_dbl_col8/61(real_back15)
  fir_dbl_col9/62(imag_back_out15) -> fir_dbl_col8/62(imag_back15)
  fir_dbl_col9/63(real_back_out16) -> fir_dbl_col8/63(real_back16)
  fir_dbl_col9/64(imag_back_out16) -> fir_dbl_col8/64(imag_back16)
  fir_dbl_col10/33(real_back_out1) -> fir_dbl_col9/33(real_back1)
  fir_dbl_col10/34(imag_back_out1) -> fir_dbl_col9/34(imag_back1)
  fir_dbl_col10/35(real_back_out2) -> fir_dbl_col9/35(real_back2)
  fir_dbl_col10/36(imag_back_out2) -> fir_dbl_col9/36(imag_back2)
  fir_dbl_col10/37(real_back_out3) -> fir_dbl_col9/37(real_back3)
  fir_dbl_col10/38(imag_back_out3) -> fir_dbl_col9/38(imag_back3)
  fir_dbl_col10/39(real_back_out4) -> fir_dbl_col9/39(real_back4)
  fir_dbl_col10/40(imag_back_out4) -> fir_dbl_col9/40(imag_back4)
  fir_dbl_col10/41(real_back_out5) -> fir_dbl_col9/41(real_back5)
  fir_dbl_col10/42(imag_back_out5) -> fir_dbl_col9/42(imag_back5)
  fir_dbl_col10/43(real_back_out6) -> fir_dbl_col9/43(real_back6)
  fir_dbl_col10/44(imag_back_out6) -> fir_dbl_col9/44(imag_back6)
  fir_dbl_col10/45(real_back_out7) -> fir_dbl_col9/45(real_back7)
  fir_dbl_col10/46(imag_back_out7) -> fir_dbl_col9/46(imag_back7)
  fir_dbl_col10/47(real_back_out8) -> fir_dbl_col9/47(real_back8)
  fir_dbl_col10/48(imag_back_out8) -> fir_dbl_col9/48(imag_back8)
  fir_dbl_col10/49(real_back_out9) -> fir_dbl_col9/49(real_back9)
  fir_dbl_col10/50(imag_back_out9) -> fir_dbl_col9/50(imag_back9)
  fir_dbl_col10/51(real_back_out10) -> fir_dbl_col9/51(real_back10)
  fir_dbl_col10/52(imag_back_out10) -> fir_dbl_col9/52(imag_back10)
  fir_dbl_col10/53(real_back_out11) -> fir_dbl_col9/53(real_back11)
  fir_dbl_col10/54(imag_back_out11) -> fir_dbl_col9/54(imag_back11)
  fir_dbl_col10/55(real_back_out12) -> fir_dbl_col9/55(real_back12)
  fir_dbl_col10/56(imag_back_out12) -> fir_dbl_col9/56(imag_back12)
  fir_dbl_col10/57(real_back_out13) -> fir_dbl_col9/57(real_back13)
  fir_dbl_col10/58(imag_back_out13) -> fir_dbl_col9/58(imag_back13)
  fir_dbl_col10/59(real_back_out14) -> fir_dbl_col9/59(real_back14)
  fir_dbl_col10/60(imag_back_out14) -> fir_dbl_col9/60(imag_back14)
  fir_dbl_col10/61(real_back_out15) -> fir_dbl_col9/61(real_back15)
  fir_dbl_col10/62(imag_back_out15) -> fir_dbl_col9/62(imag_back15)
  fir_dbl_col10/63(real_back_out16) -> fir_dbl_col9/63(real_back16)
  fir_dbl_col10/64(imag_back_out16) -> fir_dbl_col9/64(imag_back16)
  fir_dbl_col11/33(real_back_out1) -> fir_dbl_col10/33(real_back1)
  fir_dbl_col11/34(imag_back_out1) -> fir_dbl_col10/34(imag_back1)
  fir_dbl_col11/35(real_back_out2) -> fir_dbl_col10/35(real_back2)
  fir_dbl_col11/36(imag_back_out2) -> fir_dbl_col10/36(imag_back2)
  fir_dbl_col11/37(real_back_out3) -> fir_dbl_col10/37(real_back3)
  fir_dbl_col11/38(imag_back_out3) -> fir_dbl_col10/38(imag_back3)
  fir_dbl_col11/39(real_back_out4) -> fir_dbl_col10/39(real_back4)
  fir_dbl_col11/40(imag_back_out4) -> fir_dbl_col10/40(imag_back4)
  fir_dbl_col11/41(real_back_out5) -> fir_dbl_col10/41(real_back5)
  fir_dbl_col11/42(imag_back_out5) -> fir_dbl_col10/42(imag_back5)
  fir_dbl_col11/43(real_back_out6) -> fir_dbl_col10/43(real_back6)
  fir_dbl_col11/44(imag_back_out6) -> fir_dbl_col10/44(imag_back6)
  fir_dbl_col11/45(real_back_out7) -> fir_dbl_col10/45(real_back7)
  fir_dbl_col11/46(imag_back_out7) -> fir_dbl_col10/46(imag_back7)
  fir_dbl_col11/47(real_back_out8) -> fir_dbl_col10/47(real_back8)
  fir_dbl_col11/48(imag_back_out8) -> fir_dbl_col10/48(imag_back8)
  fir_dbl_col11/49(real_back_out9) -> fir_dbl_col10/49(real_back9)
  fir_dbl_col11/50(imag_back_out9) -> fir_dbl_col10/50(imag_back9)
  fir_dbl_col11/51(real_back_out10) -> fir_dbl_col10/51(real_back10)
  fir_dbl_col11/52(imag_back_out10) -> fir_dbl_col10/52(imag_back10)
  fir_dbl_col11/53(real_back_out11) -> fir_dbl_col10/53(real_back11)
  fir_dbl_col11/54(imag_back_out11) -> fir_dbl_col10/54(imag_back11)
  fir_dbl_col11/55(real_back_out12) -> fir_dbl_col10/55(real_back12)
  fir_dbl_col11/56(imag_back_out12) -> fir_dbl_col10/56(imag_back12)
  fir_dbl_col11/57(real_back_out13) -> fir_dbl_col10/57(real_back13)
  fir_dbl_col11/58(imag_back_out13) -> fir_dbl_col10/58(imag_back13)
  fir_dbl_col11/59(real_back_out14) -> fir_dbl_col10/59(real_back14)
  fir_dbl_col11/60(imag_back_out14) -> fir_dbl_col10/60(imag_back14)
  fir_dbl_col11/61(real_back_out15) -> fir_dbl_col10/61(real_back15)
  fir_dbl_col11/62(imag_back_out15) -> fir_dbl_col10/62(imag_back15)
  fir_dbl_col11/63(real_back_out16) -> fir_dbl_col10/63(real_back16)
  fir_dbl_col11/64(imag_back_out16) -> fir_dbl_col10/64(imag_back16)
  fir_dbl_col12/33(real_back_out1) -> fir_dbl_col11/33(real_back1)
  fir_dbl_col12/34(imag_back_out1) -> fir_dbl_col11/34(imag_back1)
  fir_dbl_col12/35(real_back_out2) -> fir_dbl_col11/35(real_back2)
  fir_dbl_col12/36(imag_back_out2) -> fir_dbl_col11/36(imag_back2)
  fir_dbl_col12/37(real_back_out3) -> fir_dbl_col11/37(real_back3)
  fir_dbl_col12/38(imag_back_out3) -> fir_dbl_col11/38(imag_back3)
  fir_dbl_col12/39(real_back_out4) -> fir_dbl_col11/39(real_back4)
  fir_dbl_col12/40(imag_back_out4) -> fir_dbl_col11/40(imag_back4)
  fir_dbl_col12/41(real_back_out5) -> fir_dbl_col11/41(real_back5)
  fir_dbl_col12/42(imag_back_out5) -> fir_dbl_col11/42(imag_back5)
  fir_dbl_col12/43(real_back_out6) -> fir_dbl_col11/43(real_back6)
  fir_dbl_col12/44(imag_back_out6) -> fir_dbl_col11/44(imag_back6)
  fir_dbl_col12/45(real_back_out7) -> fir_dbl_col11/45(real_back7)
  fir_dbl_col12/46(imag_back_out7) -> fir_dbl_col11/46(imag_back7)
  fir_dbl_col12/47(real_back_out8) -> fir_dbl_col11/47(real_back8)
  fir_dbl_col12/48(imag_back_out8) -> fir_dbl_col11/48(imag_back8)
  fir_dbl_col12/49(real_back_out9) -> fir_dbl_col11/49(real_back9)
  fir_dbl_col12/50(imag_back_out9) -> fir_dbl_col11/50(imag_back9)
  fir_dbl_col12/51(real_back_out10) -> fir_dbl_col11/51(real_back10)
  fir_dbl_col12/52(imag_back_out10) -> fir_dbl_col11/52(imag_back10)
  fir_dbl_col12/53(real_back_out11) -> fir_dbl_col11/53(real_back11)
  fir_dbl_col12/54(imag_back_out11) -> fir_dbl_col11/54(imag_back11)
  fir_dbl_col12/55(real_back_out12) -> fir_dbl_col11/55(real_back12)
  fir_dbl_col12/56(imag_back_out12) -> fir_dbl_col11/56(imag_back12)
  fir_dbl_col12/57(real_back_out13) -> fir_dbl_col11/57(real_back13)
  fir_dbl_col12/58(imag_back_out13) -> fir_dbl_col11/58(imag_back13)
  fir_dbl_col12/59(real_back_out14) -> fir_dbl_col11/59(real_back14)
  fir_dbl_col12/60(imag_back_out14) -> fir_dbl_col11/60(imag_back14)
  fir_dbl_col12/61(real_back_out15) -> fir_dbl_col11/61(real_back15)
  fir_dbl_col12/62(imag_back_out15) -> fir_dbl_col11/62(imag_back15)
  fir_dbl_col12/63(real_back_out16) -> fir_dbl_col11/63(real_back16)
  fir_dbl_col12/64(imag_back_out16) -> fir_dbl_col11/64(imag_back16)
  fir_dbl_col13/33(real_back_out1) -> fir_dbl_col12/33(real_back1)
  fir_dbl_col13/34(imag_back_out1) -> fir_dbl_col12/34(imag_back1)
  fir_dbl_col13/35(real_back_out2) -> fir_dbl_col12/35(real_back2)
  fir_dbl_col13/36(imag_back_out2) -> fir_dbl_col12/36(imag_back2)
  fir_dbl_col13/37(real_back_out3) -> fir_dbl_col12/37(real_back3)
  fir_dbl_col13/38(imag_back_out3) -> fir_dbl_col12/38(imag_back3)
  fir_dbl_col13/39(real_back_out4) -> fir_dbl_col12/39(real_back4)
  fir_dbl_col13/40(imag_back_out4) -> fir_dbl_col12/40(imag_back4)
  fir_dbl_col13/41(real_back_out5) -> fir_dbl_col12/41(real_back5)
  fir_dbl_col13/42(imag_back_out5) -> fir_dbl_col12/42(imag_back5)
  fir_dbl_col13/43(real_back_out6) -> fir_dbl_col12/43(real_back6)
  fir_dbl_col13/44(imag_back_out6) -> fir_dbl_col12/44(imag_back6)
  fir_dbl_col13/45(real_back_out7) -> fir_dbl_col12/45(real_back7)
  fir_dbl_col13/46(imag_back_out7) -> fir_dbl_col12/46(imag_back7)
  fir_dbl_col13/47(real_back_out8) -> fir_dbl_col12/47(real_back8)
  fir_dbl_col13/48(imag_back_out8) -> fir_dbl_col12/48(imag_back8)
  fir_dbl_col13/49(real_back_out9) -> fir_dbl_col12/49(real_back9)
  fir_dbl_col13/50(imag_back_out9) -> fir_dbl_col12/50(imag_back9)
  fir_dbl_col13/51(real_back_out10) -> fir_dbl_col12/51(real_back10)
  fir_dbl_col13/52(imag_back_out10) -> fir_dbl_col12/52(imag_back10)
  fir_dbl_col13/53(real_back_out11) -> fir_dbl_col12/53(real_back11)
  fir_dbl_col13/54(imag_back_out11) -> fir_dbl_col12/54(imag_back11)
  fir_dbl_col13/55(real_back_out12) -> fir_dbl_col12/55(real_back12)
  fir_dbl_col13/56(imag_back_out12) -> fir_dbl_col12/56(imag_back12)
  fir_dbl_col13/57(real_back_out13) -> fir_dbl_col12/57(real_back13)
  fir_dbl_col13/58(imag_back_out13) -> fir_dbl_col12/58(imag_back13)
  fir_dbl_col13/59(real_back_out14) -> fir_dbl_col12/59(real_back14)
  fir_dbl_col13/60(imag_back_out14) -> fir_dbl_col12/60(imag_back14)
  fir_dbl_col13/61(real_back_out15) -> fir_dbl_col12/61(real_back15)
  fir_dbl_col13/62(imag_back_out15) -> fir_dbl_col12/62(imag_back15)
  fir_dbl_col13/63(real_back_out16) -> fir_dbl_col12/63(real_back16)
  fir_dbl_col13/64(imag_back_out16) -> fir_dbl_col12/64(imag_back16)
  fir_dbl_col14/33(real_back_out1) -> fir_dbl_col13/33(real_back1)
  fir_dbl_col14/34(imag_back_out1) -> fir_dbl_col13/34(imag_back1)
  fir_dbl_col14/35(real_back_out2) -> fir_dbl_col13/35(real_back2)
  fir_dbl_col14/36(imag_back_out2) -> fir_dbl_col13/36(imag_back2)
  fir_dbl_col14/37(real_back_out3) -> fir_dbl_col13/37(real_back3)
  fir_dbl_col14/38(imag_back_out3) -> fir_dbl_col13/38(imag_back3)
  fir_dbl_col14/39(real_back_out4) -> fir_dbl_col13/39(real_back4)
  fir_dbl_col14/40(imag_back_out4) -> fir_dbl_col13/40(imag_back4)
  fir_dbl_col14/41(real_back_out5) -> fir_dbl_col13/41(real_back5)
  fir_dbl_col14/42(imag_back_out5) -> fir_dbl_col13/42(imag_back5)
  fir_dbl_col14/43(real_back_out6) -> fir_dbl_col13/43(real_back6)
  fir_dbl_col14/44(imag_back_out6) -> fir_dbl_col13/44(imag_back6)
  fir_dbl_col14/45(real_back_out7) -> fir_dbl_col13/45(real_back7)
  fir_dbl_col14/46(imag_back_out7) -> fir_dbl_col13/46(imag_back7)
  fir_dbl_col14/47(real_back_out8) -> fir_dbl_col13/47(real_back8)
  fir_dbl_col14/48(imag_back_out8) -> fir_dbl_col13/48(imag_back8)
  fir_dbl_col14/49(real_back_out9) -> fir_dbl_col13/49(real_back9)
  fir_dbl_col14/50(imag_back_out9) -> fir_dbl_col13/50(imag_back9)
  fir_dbl_col14/51(real_back_out10) -> fir_dbl_col13/51(real_back10)
  fir_dbl_col14/52(imag_back_out10) -> fir_dbl_col13/52(imag_back10)
  fir_dbl_col14/53(real_back_out11) -> fir_dbl_col13/53(real_back11)
  fir_dbl_col14/54(imag_back_out11) -> fir_dbl_col13/54(imag_back11)
  fir_dbl_col14/55(real_back_out12) -> fir_dbl_col13/55(real_back12)
  fir_dbl_col14/56(imag_back_out12) -> fir_dbl_col13/56(imag_back12)
  fir_dbl_col14/57(real_back_out13) -> fir_dbl_col13/57(real_back13)
  fir_dbl_col14/58(imag_back_out13) -> fir_dbl_col13/58(imag_back13)
  fir_dbl_col14/59(real_back_out14) -> fir_dbl_col13/59(real_back14)
  fir_dbl_col14/60(imag_back_out14) -> fir_dbl_col13/60(imag_back14)
  fir_dbl_col14/61(real_back_out15) -> fir_dbl_col13/61(real_back15)
  fir_dbl_col14/62(imag_back_out15) -> fir_dbl_col13/62(imag_back15)
  fir_dbl_col14/63(real_back_out16) -> fir_dbl_col13/63(real_back16)
  fir_dbl_col14/64(imag_back_out16) -> fir_dbl_col13/64(imag_back16)
  fir_dbl_col15/33(real_back_out1) -> fir_dbl_col14/33(real_back1)
  fir_dbl_col15/34(imag_back_out1) -> fir_dbl_col14/34(imag_back1)
  fir_dbl_col15/35(real_back_out2) -> fir_dbl_col14/35(real_back2)
  fir_dbl_col15/36(imag_back_out2) -> fir_dbl_col14/36(imag_back2)
  fir_dbl_col15/37(real_back_out3) -> fir_dbl_col14/37(real_back3)
  fir_dbl_col15/38(imag_back_out3) -> fir_dbl_col14/38(imag_back3)
  fir_dbl_col15/39(real_back_out4) -> fir_dbl_col14/39(real_back4)
  fir_dbl_col15/40(imag_back_out4) -> fir_dbl_col14/40(imag_back4)
  fir_dbl_col15/41(real_back_out5) -> fir_dbl_col14/41(real_back5)
  fir_dbl_col15/42(imag_back_out5) -> fir_dbl_col14/42(imag_back5)
  fir_dbl_col15/43(real_back_out6) -> fir_dbl_col14/43(real_back6)
  fir_dbl_col15/44(imag_back_out6) -> fir_dbl_col14/44(imag_back6)
  fir_dbl_col15/45(real_back_out7) -> fir_dbl_col14/45(real_back7)
  fir_dbl_col15/46(imag_back_out7) -> fir_dbl_col14/46(imag_back7)
  fir_dbl_col15/47(real_back_out8) -> fir_dbl_col14/47(real_back8)
  fir_dbl_col15/48(imag_back_out8) -> fir_dbl_col14/48(imag_back8)
  fir_dbl_col15/49(real_back_out9) -> fir_dbl_col14/49(real_back9)
  fir_dbl_col15/50(imag_back_out9) -> fir_dbl_col14/50(imag_back9)
  fir_dbl_col15/51(real_back_out10) -> fir_dbl_col14/51(real_back10)
  fir_dbl_col15/52(imag_back_out10) -> fir_dbl_col14/52(imag_back10)
  fir_dbl_col15/53(real_back_out11) -> fir_dbl_col14/53(real_back11)
  fir_dbl_col15/54(imag_back_out11) -> fir_dbl_col14/54(imag_back11)
  fir_dbl_col15/55(real_back_out12) -> fir_dbl_col14/55(real_back12)
  fir_dbl_col15/56(imag_back_out12) -> fir_dbl_col14/56(imag_back12)
  fir_dbl_col15/57(real_back_out13) -> fir_dbl_col14/57(real_back13)
  fir_dbl_col15/58(imag_back_out13) -> fir_dbl_col14/58(imag_back13)
  fir_dbl_col15/59(real_back_out14) -> fir_dbl_col14/59(real_back14)
  fir_dbl_col15/60(imag_back_out14) -> fir_dbl_col14/60(imag_back14)
  fir_dbl_col15/61(real_back_out15) -> fir_dbl_col14/61(real_back15)
  fir_dbl_col15/62(imag_back_out15) -> fir_dbl_col14/62(imag_back15)
  fir_dbl_col15/63(real_back_out16) -> fir_dbl_col14/63(real_back16)
  fir_dbl_col15/64(imag_back_out16) -> fir_dbl_col14/64(imag_back16)
  fir_dbl_col16/33(real_back_out1) -> fir_dbl_col15/33(real_back1)
  fir_dbl_col16/34(imag_back_out1) -> fir_dbl_col15/34(imag_back1)
  fir_dbl_col16/35(real_back_out2) -> fir_dbl_col15/35(real_back2)
  fir_dbl_col16/36(imag_back_out2) -> fir_dbl_col15/36(imag_back2)
  fir_dbl_col16/37(real_back_out3) -> fir_dbl_col15/37(real_back3)
  fir_dbl_col16/38(imag_back_out3) -> fir_dbl_col15/38(imag_back3)
  fir_dbl_col16/39(real_back_out4) -> fir_dbl_col15/39(real_back4)
  fir_dbl_col16/40(imag_back_out4) -> fir_dbl_col15/40(imag_back4)
  fir_dbl_col16/41(real_back_out5) -> fir_dbl_col15/41(real_back5)
  fir_dbl_col16/42(imag_back_out5) -> fir_dbl_col15/42(imag_back5)
  fir_dbl_col16/43(real_back_out6) -> fir_dbl_col15/43(real_back6)
  fir_dbl_col16/44(imag_back_out6) -> fir_dbl_col15/44(imag_back6)
  fir_dbl_col16/45(real_back_out7) -> fir_dbl_col15/45(real_back7)
  fir_dbl_col16/46(imag_back_out7) -> fir_dbl_col15/46(imag_back7)
  fir_dbl_col16/47(real_back_out8) -> fir_dbl_col15/47(real_back8)
  fir_dbl_col16/48(imag_back_out8) -> fir_dbl_col15/48(imag_back8)
  fir_dbl_col16/49(real_back_out9) -> fir_dbl_col15/49(real_back9)
  fir_dbl_col16/50(imag_back_out9) -> fir_dbl_col15/50(imag_back9)
  fir_dbl_col16/51(real_back_out10) -> fir_dbl_col15/51(real_back10)
  fir_dbl_col16/52(imag_back_out10) -> fir_dbl_col15/52(imag_back10)
  fir_dbl_col16/53(real_back_out11) -> fir_dbl_col15/53(real_back11)
  fir_dbl_col16/54(imag_back_out11) -> fir_dbl_col15/54(imag_back11)
  fir_dbl_col16/55(real_back_out12) -> fir_dbl_col15/55(real_back12)
  fir_dbl_col16/56(imag_back_out12) -> fir_dbl_col15/56(imag_back12)
  fir_dbl_col16/57(real_back_out13) -> fir_dbl_col15/57(real_back13)
  fir_dbl_col16/58(imag_back_out13) -> fir_dbl_col15/58(imag_back13)
  fir_dbl_col16/59(real_back_out14) -> fir_dbl_col15/59(real_back14)
  fir_dbl_col16/60(imag_back_out14) -> fir_dbl_col15/60(imag_back14)
  fir_dbl_col16/61(real_back_out15) -> fir_dbl_col15/61(real_back15)
  fir_dbl_col16/62(imag_back_out15) -> fir_dbl_col15/62(imag_back15)
  fir_dbl_col16/63(real_back_out16) -> fir_dbl_col15/63(real_back16)
  fir_dbl_col16/64(imag_back_out16) -> fir_dbl_col15/64(imag_back16)
  fir_dbl_col16/1(real_out1) -> fir_dbl_col16/33(real_back1)
  fir_dbl_col16/2(imag_out1) -> fir_dbl_col16/34(imag_back1)
  fir_dbl_col16/3(real_out2) -> fir_dbl_col16/35(real_back2)
  fir_dbl_col16/4(imag_out2) -> fir_dbl_col16/36(imag_back2)
  fir_dbl_col16/5(real_out3) -> fir_dbl_col16/37(real_back3)
  fir_dbl_col16/6(imag_out3) -> fir_dbl_col16/38(imag_back3)
  fir_dbl_col16/7(real_out4) -> fir_dbl_col16/39(real_back4)
  fir_dbl_col16/8(imag_out4) -> fir_dbl_col16/40(imag_back4)
  fir_dbl_col16/9(real_out5) -> fir_dbl_col16/41(real_back5)
  fir_dbl_col16/10(imag_out5) -> fir_dbl_col16/42(imag_back5)
  fir_dbl_col16/11(real_out6) -> fir_dbl_col16/43(real_back6)
  fir_dbl_col16/12(imag_out6) -> fir_dbl_col16/44(imag_back6)
  fir_dbl_col16/13(real_out7) -> fir_dbl_col16/45(real_back7)
  fir_dbl_col16/14(imag_out7) -> fir_dbl_col16/46(imag_back7)
  fir_dbl_col16/15(real_out8) -> fir_dbl_col16/47(real_back8)
  fir_dbl_col16/16(imag_out8) -> fir_dbl_col16/48(imag_back8)
  fir_dbl_col16/17(real_out9) -> fir_dbl_col16/49(real_back9)
  fir_dbl_col16/18(imag_out9) -> fir_dbl_col16/50(imag_back9)
  fir_dbl_col16/19(real_out10) -> fir_dbl_col16/51(real_back10)
  fir_dbl_col16/20(imag_out10) -> fir_dbl_col16/52(imag_back10)
  fir_dbl_col16/21(real_out11) -> fir_dbl_col16/53(real_back11)
  fir_dbl_col16/22(imag_out11) -> fir_dbl_col16/54(imag_back11)
  fir_dbl_col16/23(real_out12) -> fir_dbl_col16/55(real_back12)
  fir_dbl_col16/24(imag_out12) -> fir_dbl_col16/56(imag_back12)
  fir_dbl_col16/25(real_out13) -> fir_dbl_col16/57(real_back13)
  fir_dbl_col16/26(imag_out13) -> fir_dbl_col16/58(imag_back13)
  fir_dbl_col16/27(real_out14) -> fir_dbl_col16/59(real_back14)
  fir_dbl_col16/28(imag_out14) -> fir_dbl_col16/60(imag_back14)
  fir_dbl_col16/29(real_out15) -> fir_dbl_col16/61(real_back15)
  fir_dbl_col16/30(imag_out15) -> fir_dbl_col16/62(imag_back15)
  fir_dbl_col16/31(real_out16) -> fir_dbl_col16/63(real_back16)
  fir_dbl_col16/32(imag_out16) -> fir_dbl_col16/64(imag_back16)
